simulink model "model_compatible"  (Simulink 7.5)
(part 8 of 10)

      | %<Name>
  bus795 : powerlib/Measurements/Load Flow Bus  LConnTagsString=a  Phases=single  Connectors=on one side  ID=bus795  Vbase=380000  Vref=1  Vangle=0  VLF=1  VLFb=1  VLFc=1  angleLF=0  angleLFb=0  angleLFc=0
      settings: AttributesFormatString=|
      | %<ID>
      | %<Vbase>V
      | %<VLF>pu
      | %<angleLF>deg.
      | %<Name>
  bus796 : powerlib/Measurements/Load Flow Bus  LConnTagsString=a  Phases=single  Connectors=on one side  ID=bus796  Vbase=380000  Vref=1  Vangle=0  VLF=1  VLFb=1  VLFc=1  angleLF=0  angleLFb=0  angleLFc=0
      settings: AttributesFormatString=|
      | %<ID>
      | %<Vbase>V
      | %<VLF>pu
      | %<angleLF>deg.
      | %<Name>
  bus797 : powerlib/Measurements/Load Flow Bus  LConnTagsString=a  Phases=single  Connectors=on one side  ID=bus797  Vbase=380000  Vref=1  Vangle=0  VLF=1  VLFb=1  VLFc=1  angleLF=0  angleLFb=0  angleLFc=0
      settings: AttributesFormatString=|
      | %<ID>
      | %<Vbase>V
      | %<VLF>pu
      | %<angleLF>deg.
      | %<Name>
  bus798 : powerlib/Measurements/Load Flow Bus  LConnTagsString=a  Phases=single  Connectors=on one side  ID=bus798  Vbase=380000  Vref=1  Vangle=0  VLF=1  VLFb=1  VLFc=1  angleLF=0  angleLFb=0  angleLFc=0
      settings: AttributesFormatString=|
      | %<ID>
      | %<Vbase>V
      | %<VLF>pu
      | %<angleLF>deg.
      | %<Name>
  bus799 : powerlib/Measurements/Load Flow Bus  LConnTagsString=a  Phases=single  Connectors=on one side  ID=bus799  Vbase=380000  Vref=1  Vangle=0  VLF=1  VLFb=1  VLFc=1  angleLF=0  angleLFb=0  angleLFc=0
      settings: AttributesFormatString=|
      | %<ID>
      | %<Vbase>V
      | %<VLF>pu
      | %<angleLF>deg.
      | %<Name>
  bus8 : powerlib/Measurements/Load Flow Bus  LConnTagsString=a  Phases=single  Connectors=on one side  ID=bus8  Vbase=220000  Vref=1  Vangle=0  VLF=1  VLFb=1  VLFc=1  angleLF=0  angleLFb=0  angleLFc=0
      settings: AttributesFormatString=|
      | %<ID>
      | %<Vbase>V
      | %<VLF>pu
      | %<angleLF>deg.
      | %<Name>
  bus80 : powerlib/Measurements/Load Flow Bus  LConnTagsString=a  Phases=single  Connectors=on one side  ID=bus80  Vbase=220000  Vref=1  Vangle=0  VLF=1  VLFb=1  VLFc=1  angleLF=0  angleLFb=0  angleLFc=0
      settings: AttributesFormatString=|
      | %<ID>
      | %<Vbase>V
      | %<VLF>pu
      | %<angleLF>deg.
      | %<Name>
  bus800 : powerlib/Measurements/Load Flow Bus  LConnTagsString=a  Phases=single  Connectors=on one side  ID=bus800  Vbase=380000  Vref=1  Vangle=0  VLF=1  VLFb=1  VLFc=1  angleLF=0  angleLFb=0  angleLFc=0
      settings: AttributesFormatString=|
      | %<ID>
      | %<Vbase>V
      | %<VLF>pu
      | %<angleLF>deg.
      | %<Name>
  bus801 : powerlib/Measurements/Load Flow Bus  LConnTagsString=a  Phases=single  Connectors=on one side  ID=bus801  Vbase=380000  Vref=1  Vangle=0  VLF=1  VLFb=1  VLFc=1  angleLF=0  angleLFb=0  angleLFc=0
      settings: AttributesFormatString=|
      | %<ID>
      | %<Vbase>V
      | %<VLF>pu
      | %<angleLF>deg.
      | %<Name>
  bus802 : powerlib/Measurements/Load Flow Bus  LConnTagsString=a  Phases=single  Connectors=on one side  ID=bus802  Vbase=380000  Vref=1  Vangle=0  VLF=1  VLFb=1  VLFc=1  angleLF=0  angleLFb=0  angleLFc=0
      settings: AttributesFormatString=|
      | %<ID>
      | %<Vbase>V
      | %<VLF>pu
      | %<angleLF>deg.
      | %<Name>
  bus803 : powerlib/Measurements/Load Flow Bus  LConnTagsString=a  Phases=single  Connectors=on one side  ID=bus803  Vbase=380000  Vref=1  Vangle=0  VLF=1  VLFb=1  VLFc=1  angleLF=0  angleLFb=0  angleLFc=0
      settings: AttributesFormatString=|
      | %<ID>
      | %<Vbase>V
      | %<VLF>pu
      | %<angleLF>deg.
      | %<Name>
  bus804 : powerlib/Measurements/Load Flow Bus  LConnTagsString=a  Phases=single  Connectors=on one side  ID=bus804  Vbase=380000  Vref=1  Vangle=0  VLF=1  VLFb=1  VLFc=1  angleLF=0  angleLFb=0  angleLFc=0
      settings: AttributesFormatString=|
      | %<ID>
      | %<Vbase>V
      | %<VLF>pu
      | %<angleLF>deg.
      | %<Name>
  bus805 : powerlib/Measurements/Load Flow Bus  LConnTagsString=a  Phases=single  Connectors=on one side  ID=bus805  Vbase=380000  Vref=1  Vangle=0  VLF=1  VLFb=1  VLFc=1  angleLF=0  angleLFb=0  angleLFc=0
      settings: AttributesFormatString=|
      | %<ID>
      | %<Vbase>V
      | %<VLF>pu
      | %<angleLF>deg.
      | %<Name>
  bus806 : powerlib/Measurements/Load Flow Bus  LConnTagsString=a  Phases=single  Connectors=on one side  ID=bus806  Vbase=380000  Vref=1  Vangle=0  VLF=1  VLFb=1  VLFc=1  angleLF=0  angleLFb=0  angleLFc=0
      settings: AttributesFormatString=|
      | %<ID>
      | %<Vbase>V
      | %<VLF>pu
      | %<angleLF>deg.
      | %<Name>
  bus807 : powerlib/Measurements/Load Flow Bus  LConnTagsString=a  Phases=single  Connectors=on one side  ID=bus807  Vbase=380000  Vref=1  Vangle=0  VLF=1  VLFb=1  VLFc=1  angleLF=0  angleLFb=0  angleLFc=0
      settings: AttributesFormatString=|
      | %<ID>
      | %<Vbase>V
      | %<VLF>pu
      | %<angleLF>deg.
      | %<Name>
  bus808 : powerlib/Measurements/Load Flow Bus  LConnTagsString=a  Phases=single  Connectors=on one side  ID=bus808  Vbase=380000  Vref=1  Vangle=0  VLF=1  VLFb=1  VLFc=1  angleLF=0  angleLFb=0  angleLFc=0
      settings: AttributesFormatString=|
      | %<ID>
      | %<Vbase>V
      | %<VLF>pu
      | %<angleLF>deg.
      | %<Name>
  bus809 : powerlib/Measurements/Load Flow Bus  LConnTagsString=a  Phases=single  Connectors=on one side  ID=bus809  Vbase=132000  Vref=1  Vangle=0  VLF=1  VLFb=1  VLFc=1  angleLF=0  angleLFb=0  angleLFc=0
      settings: AttributesFormatString=|
      | %<ID>
      | %<Vbase>V
      | %<VLF>pu
      | %<angleLF>deg.
      | %<Name>
  bus81 : powerlib/Measurements/Load Flow Bus  LConnTagsString=a  Phases=single  Connectors=on one side  ID=bus81  Vbase=220000  Vref=1  Vangle=0  VLF=1  VLFb=1  VLFc=1  angleLF=0  angleLFb=0  angleLFc=0
      settings: AttributesFormatString=|
      | %<ID>
      | %<Vbase>V
      | %<VLF>pu
      | %<angleLF>deg.
      | %<Name>
  bus810 : powerlib/Measurements/Load Flow Bus  LConnTagsString=a  Phases=single  Connectors=on one side  ID=bus810  Vbase=380000  Vref=1  Vangle=0  VLF=1  VLFb=1  VLFc=1  angleLF=0  angleLFb=0  angleLFc=0
      settings: AttributesFormatString=|
      | %<ID>
      | %<Vbase>V
      | %<VLF>pu
      | %<angleLF>deg.
      | %<Name>
  bus811 : powerlib/Measurements/Load Flow Bus  LConnTagsString=a  Phases=single  Connectors=on one side  ID=bus811  Vbase=380000  Vref=1  Vangle=0  VLF=1  VLFb=1  VLFc=1  angleLF=0  angleLFb=0  angleLFc=0
      settings: AttributesFormatString=|
      | %<ID>
      | %<Vbase>V
      | %<VLF>pu
      | %<angleLF>deg.
      | %<Name>
  bus812 : powerlib/Measurements/Load Flow Bus  LConnTagsString=a  Phases=single  Connectors=on one side  ID=bus812  Vbase=380000  Vref=1  Vangle=0  VLF=1  VLFb=1  VLFc=1  angleLF=0  angleLFb=0  angleLFc=0
      settings: AttributesFormatString=|
      | %<ID>
      | %<Vbase>V
      | %<VLF>pu
      | %<angleLF>deg.
      | %<Name>
  bus813 : powerlib/Measurements/Load Flow Bus  LConnTagsString=a  Phases=single  Connectors=on one side  ID=bus813  Vbase=380000  Vref=1  Vangle=0  VLF=1  VLFb=1  VLFc=1  angleLF=0  angleLFb=0  angleLFc=0
      settings: AttributesFormatString=|
      | %<ID>
      | %<Vbase>V
      | %<VLF>pu
      | %<angleLF>deg.
      | %<Name>
  bus814 : powerlib/Measurements/Load Flow Bus  LConnTagsString=a  Phases=single  Connectors=on one side  ID=bus814  Vbase=380000  Vref=1  Vangle=0  VLF=1  VLFb=1  VLFc=1  angleLF=0  angleLFb=0  angleLFc=0
      settings: AttributesFormatString=|
      | %<ID>
      | %<Vbase>V
      | %<VLF>pu
      | %<angleLF>deg.
      | %<Name>
  bus815 : powerlib/Measurements/Load Flow Bus  LConnTagsString=a  Phases=single  Connectors=on one side  ID=bus815  Vbase=380000  Vref=1  Vangle=0  VLF=1  VLFb=1  VLFc=1  angleLF=0  angleLFb=0  angleLFc=0
      settings: AttributesFormatString=|
      | %<ID>
      | %<Vbase>V
      | %<VLF>pu
      | %<angleLF>deg.
      | %<Name>
  bus816 : powerlib/Measurements/Load Flow Bus  LConnTagsString=a  Phases=single  Connectors=on one side  ID=bus816  Vbase=380000  Vref=1  Vangle=0  VLF=1  VLFb=1  VLFc=1  angleLF=0  angleLFb=0  angleLFc=0
      settings: AttributesFormatString=|
      | %<ID>
      | %<Vbase>V
      | %<VLF>pu
      | %<angleLF>deg.
      | %<Name>
  bus817 : powerlib/Measurements/Load Flow Bus  LConnTagsString=a  Phases=single  Connectors=on one side  ID=bus817  Vbase=380000  Vref=1  Vangle=0  VLF=1  VLFb=1  VLFc=1  angleLF=0  angleLFb=0  angleLFc=0
      settings: AttributesFormatString=|
      | %<ID>
      | %<Vbase>V
      | %<VLF>pu
      | %<angleLF>deg.
      | %<Name>
  bus818 : powerlib/Measurements/Load Flow Bus  LConnTagsString=a  Phases=single  Connectors=on one side  ID=bus818  Vbase=380000  Vref=1  Vangle=0  VLF=1  VLFb=1  VLFc=1  angleLF=0  angleLFb=0  angleLFc=0
      settings: AttributesFormatString=|
      | %<ID>
      | %<Vbase>V
      | %<VLF>pu
      | %<angleLF>deg.
      | %<Name>
  bus819 : powerlib/Measurements/Load Flow Bus  LConnTagsString=a  Phases=single  Connectors=on one side  ID=bus819  Vbase=380000  Vref=1  Vangle=0  VLF=1  VLFb=1  VLFc=1  angleLF=0  angleLFb=0  angleLFc=0
      settings: AttributesFormatString=|
      | %<ID>
      | %<Vbase>V
      | %<VLF>pu
      | %<angleLF>deg.
      | %<Name>
  bus82 : powerlib/Measurements/Load Flow Bus  LConnTagsString=a  Phases=single  Connectors=on one side  ID=bus82  Vbase=220000  Vref=1  Vangle=0  VLF=1  VLFb=1  VLFc=1  angleLF=0  angleLFb=0  angleLFc=0
      settings: AttributesFormatString=|
      | %<ID>
      | %<Vbase>V
      | %<VLF>pu
      | %<angleLF>deg.
      | %<Name>
  bus820 : powerlib/Measurements/Load Flow Bus  LConnTagsString=a  Phases=single  Connectors=on one side  ID=bus820  Vbase=380000  Vref=1  Vangle=0  VLF=1  VLFb=1  VLFc=1  angleLF=0  angleLFb=0  angleLFc=0
      settings: AttributesFormatString=|
      | %<ID>
      | %<Vbase>V
      | %<VLF>pu
      | %<angleLF>deg.
      | %<Name>
  bus821 : powerlib/Measurements/Load Flow Bus  LConnTagsString=a  Phases=single  Connectors=on one side  ID=bus821  Vbase=380000  Vref=1  Vangle=0  VLF=1  VLFb=1  VLFc=1  angleLF=0  angleLFb=0  angleLFc=0
      settings: AttributesFormatString=|
      | %<ID>
      | %<Vbase>V
      | %<VLF>pu
      | %<angleLF>deg.
      | %<Name>
  bus822 : powerlib/Measurements/Load Flow Bus  LConnTagsString=a  Phases=single  Connectors=on one side  ID=bus822  Vbase=380000  Vref=1  Vangle=0  VLF=1  VLFb=1  VLFc=1  angleLF=0  angleLFb=0  angleLFc=0
      settings: AttributesFormatString=|
      | %<ID>
      | %<Vbase>V
      | %<VLF>pu
      | %<angleLF>deg.
      | %<Name>
  bus823 : powerlib/Measurements/Load Flow Bus  LConnTagsString=a  Phases=single  Connectors=on one side  ID=bus823  Vbase=380000  Vref=1  Vangle=0  VLF=1  VLFb=1  VLFc=1  angleLF=0  angleLFb=0  angleLFc=0
      settings: AttributesFormatString=|
      | %<ID>
      | %<Vbase>V
      | %<VLF>pu
      | %<angleLF>deg.
      | %<Name>
  bus824 : powerlib/Measurements/Load Flow Bus  LConnTagsString=a  Phases=single  Connectors=on one side  ID=bus824  Vbase=380000  Vref=1  Vangle=0  VLF=1  VLFb=1  VLFc=1  angleLF=0  angleLFb=0  angleLFc=0
      settings: AttributesFormatString=|
      | %<ID>
      | %<Vbase>V
      | %<VLF>pu
      | %<angleLF>deg.
      | %<Name>
  bus825 : powerlib/Measurements/Load Flow Bus  LConnTagsString=a  Phases=single  Connectors=on one side  ID=bus825  Vbase=380000  Vref=1  Vangle=0  VLF=1  VLFb=1  VLFc=1  angleLF=0  angleLFb=0  angleLFc=0
      settings: AttributesFormatString=|
      | %<ID>
      | %<Vbase>V
      | %<VLF>pu
      | %<angleLF>deg.
      | %<Name>
  bus826 : powerlib/Measurements/Load Flow Bus  LConnTagsString=a  Phases=single  Connectors=on one side  ID=bus826  Vbase=380000  Vref=1  Vangle=0  VLF=1  VLFb=1  VLFc=1  angleLF=0  angleLFb=0  angleLFc=0
      settings: AttributesFormatString=|
      | %<ID>
      | %<Vbase>V
      | %<VLF>pu
      | %<angleLF>deg.
      | %<Name>
  bus827 : powerlib/Measurements/Load Flow Bus  LConnTagsString=a  Phases=single  Connectors=on one side  ID=bus827  Vbase=380000  Vref=1  Vangle=0  VLF=1  VLFb=1  VLFc=1  angleLF=0  angleLFb=0  angleLFc=0
      settings: AttributesFormatString=|
      | %<ID>
      | %<Vbase>V
      | %<VLF>pu
      | %<angleLF>deg.
      | %<Name>
  bus828 : powerlib/Measurements/Load Flow Bus  LConnTagsString=a  Phases=single  Connectors=on one side  ID=bus828  Vbase=380000  Vref=1  Vangle=0  VLF=1  VLFb=1  VLFc=1  angleLF=0  angleLFb=0  angleLFc=0
      settings: AttributesFormatString=|
      | %<ID>
      | %<Vbase>V
      | %<VLF>pu
      | %<angleLF>deg.
      | %<Name>
  bus829 : powerlib/Measurements/Load Flow Bus  LConnTagsString=a  Phases=single  Connectors=on one side  ID=bus829  Vbase=380000  Vref=1  Vangle=0  VLF=1  VLFb=1  VLFc=1  angleLF=0  angleLFb=0  angleLFc=0
      settings: AttributesFormatString=|
      | %<ID>
      | %<Vbase>V
      | %<VLF>pu
      | %<angleLF>deg.
      | %<Name>
  bus83 : powerlib/Measurements/Load Flow Bus  LConnTagsString=a  Phases=single  Connectors=on one side  ID=bus83  Vbase=220000  Vref=1  Vangle=0  VLF=1  VLFb=1  VLFc=1  angleLF=0  angleLFb=0  angleLFc=0
      settings: AttributesFormatString=|
      | %<ID>
      | %<Vbase>V
      | %<VLF>pu
      | %<angleLF>deg.
      | %<Name>
  bus830 : powerlib/Measurements/Load Flow Bus  LConnTagsString=a  Phases=single  Connectors=on one side  ID=bus830  Vbase=380000  Vref=1  Vangle=0  VLF=1  VLFb=1  VLFc=1  angleLF=0  angleLFb=0  angleLFc=0
      settings: AttributesFormatString=|
      | %<ID>
      | %<Vbase>V
      | %<VLF>pu
      | %<angleLF>deg.
      | %<Name>
  bus831 : powerlib/Measurements/Load Flow Bus  LConnTagsString=a  Phases=single  Connectors=on one side  ID=bus831  Vbase=380000  Vref=1  Vangle=0  VLF=1  VLFb=1  VLFc=1  angleLF=0  angleLFb=0  angleLFc=0
      settings: AttributesFormatString=|
      | %<ID>
      | %<Vbase>V
      | %<VLF>pu
      | %<angleLF>deg.
      | %<Name>
  bus832 : powerlib/Measurements/Load Flow Bus  LConnTagsString=a  Phases=single  Connectors=on one side  ID=bus832  Vbase=380000  Vref=1  Vangle=0  VLF=1  VLFb=1  VLFc=1  angleLF=0  angleLFb=0  angleLFc=0
      settings: AttributesFormatString=|
      | %<ID>
      | %<Vbase>V
      | %<VLF>pu
      | %<angleLF>deg.
      | %<Name>
  bus833 : powerlib/Measurements/Load Flow Bus  LConnTagsString=a  Phases=single  Connectors=on one side  ID=bus833  Vbase=380000  Vref=1  Vangle=0  VLF=1  VLFb=1  VLFc=1  angleLF=0  angleLFb=0  angleLFc=0
      settings: AttributesFormatString=|
      | %<ID>
      | %<Vbase>V
      | %<VLF>pu
      | %<angleLF>deg.
      | %<Name>
  bus834 : powerlib/Measurements/Load Flow Bus  LConnTagsString=a  Phases=single  Connectors=on one side  ID=bus834  Vbase=380000  Vref=1  Vangle=0  VLF=1  VLFb=1  VLFc=1  angleLF=0  angleLFb=0  angleLFc=0
      settings: AttributesFormatString=|
      | %<ID>
      | %<Vbase>V
      | %<VLF>pu
      | %<angleLF>deg.
      | %<Name>
  bus835 : powerlib/Measurements/Load Flow Bus  LConnTagsString=a  Phases=single  Connectors=on one side  ID=bus835  Vbase=380000  Vref=1  Vangle=0  VLF=1  VLFb=1  VLFc=1  angleLF=0  angleLFb=0  angleLFc=0
      settings: AttributesFormatString=|
      | %<ID>
      | %<Vbase>V
      | %<VLF>pu
      | %<angleLF>deg.
      | %<Name>
  bus836 : powerlib/Measurements/Load Flow Bus  LConnTagsString=a  Phases=single  Connectors=on one side  ID=bus836  Vbase=380000  Vref=1  Vangle=0  VLF=1  VLFb=1  VLFc=1  angleLF=0  angleLFb=0  angleLFc=0
      settings: AttributesFormatString=|
      | %<ID>
      | %<Vbase>V
      | %<VLF>pu
      | %<angleLF>deg.
      | %<Name>
  bus837 : powerlib/Measurements/Load Flow Bus  LConnTagsString=a  Phases=single  Connectors=on one side  ID=bus837  Vbase=380000  Vref=1  Vangle=0  VLF=1  VLFb=1  VLFc=1  angleLF=0  angleLFb=0  angleLFc=0
      settings: AttributesFormatString=|
      | %<ID>
      | %<Vbase>V
      | %<VLF>pu
      | %<angleLF>deg.
      | %<Name>
  bus838 : powerlib/Measurements/Load Flow Bus  LConnTagsString=a  Phases=single  Connectors=on one side  ID=bus838  Vbase=380000  Vref=1  Vangle=0  VLF=1  VLFb=1  VLFc=1  angleLF=0  angleLFb=0  angleLFc=0
      settings: AttributesFormatString=|
      | %<ID>
      | %<Vbase>V
      | %<VLF>pu
      | %<angleLF>deg.
      | %<Name>
  bus839 : powerlib/Measurements/Load Flow Bus  LConnTagsString=a  Phases=single  Connectors=on one side  ID=bus839  Vbase=380000  Vref=1  Vangle=0  VLF=1  VLFb=1  VLFc=1  angleLF=0  angleLFb=0  angleLFc=0
      settings: AttributesFormatString=|
      | %<ID>
      | %<Vbase>V
      | %<VLF>pu
      | %<angleLF>deg.
      | %<Name>
  bus84 : powerlib/Measurements/Load Flow Bus  LConnTagsString=a  Phases=single  Connectors=on one side  ID=bus84  Vbase=220000  Vref=1  Vangle=0  VLF=1  VLFb=1  VLFc=1  angleLF=0  angleLFb=0  angleLFc=0
      settings: AttributesFormatString=|
      | %<ID>
      | %<Vbase>V
      | %<VLF>pu
      | %<angleLF>deg.
      | %<Name>
  bus840 : powerlib/Measurements/Load Flow Bus  LConnTagsString=a  Phases=single  Connectors=on one side  ID=bus840  Vbase=380000  Vref=1  Vangle=0  VLF=1  VLFb=1  VLFc=1  angleLF=0  angleLFb=0  angleLFc=0
      settings: AttributesFormatString=|
      | %<ID>
      | %<Vbase>V
      | %<VLF>pu
      | %<angleLF>deg.
      | %<Name>
  bus841 : powerlib/Measurements/Load Flow Bus  LConnTagsString=a  Phases=single  Connectors=on one side  ID=bus841  Vbase=380000  Vref=1  Vangle=0  VLF=1  VLFb=1  VLFc=1  angleLF=0  angleLFb=0  angleLFc=0
      settings: AttributesFormatString=|
      | %<ID>
      | %<Vbase>V
      | %<VLF>pu
      | %<angleLF>deg.
      | %<Name>
  bus842 : powerlib/Measurements/Load Flow Bus  LConnTagsString=a  Phases=single  Connectors=on one side  ID=bus842  Vbase=380000  Vref=1  Vangle=0  VLF=1  VLFb=1  VLFc=1  angleLF=0  angleLFb=0  angleLFc=0
      settings: AttributesFormatString=|
      | %<ID>
      | %<Vbase>V
      | %<VLF>pu
      | %<angleLF>deg.
      | %<Name>
  bus843 : powerlib/Measurements/Load Flow Bus  LConnTagsString=a  Phases=single  Connectors=on one side  ID=bus843  Vbase=380000  Vref=1  Vangle=0  VLF=1  VLFb=1  VLFc=1  angleLF=0  angleLFb=0  angleLFc=0
      settings: AttributesFormatString=|
      | %<ID>
      | %<Vbase>V
      | %<VLF>pu
      | %<angleLF>deg.
      | %<Name>
  bus844 : powerlib/Measurements/Load Flow Bus  LConnTagsString=a  Phases=single  Connectors=on one side  ID=bus844  Vbase=380000  Vref=1  Vangle=0  VLF=1  VLFb=1  VLFc=1  angleLF=0  angleLFb=0  angleLFc=0
      settings: AttributesFormatString=|
      | %<ID>
      | %<Vbase>V
      | %<VLF>pu
      | %<angleLF>deg.
      | %<Name>
  bus845 : powerlib/Measurements/Load Flow Bus  LConnTagsString=a  Phases=single  Connectors=on one side  ID=bus845  Vbase=380000  Vref=1  Vangle=0  VLF=1  VLFb=1  VLFc=1  angleLF=0  angleLFb=0  angleLFc=0
      settings: AttributesFormatString=|
      | %<ID>
      | %<Vbase>V
      | %<VLF>pu
      | %<angleLF>deg.
      | %<Name>
  bus846 : powerlib/Measurements/Load Flow Bus  LConnTagsString=a  Phases=single  Connectors=on one side  ID=bus846  Vbase=380000  Vref=1  Vangle=0  VLF=1  VLFb=1  VLFc=1  angleLF=0  angleLFb=0  angleLFc=0
      settings: AttributesFormatString=|
      | %<ID>
      | %<Vbase>V
      | %<VLF>pu
      | %<angleLF>deg.
      | %<Name>
  bus85 : powerlib/Measurements/Load Flow Bus  LConnTagsString=a  Phases=single  Connectors=on one side  ID=bus85  Vbase=220000  Vref=1  Vangle=0  VLF=1  VLFb=1  VLFc=1  angleLF=0  angleLFb=0  angleLFc=0
      settings: AttributesFormatString=|
      | %<ID>
      | %<Vbase>V
      | %<VLF>pu
      | %<angleLF>deg.
      | %<Name>
  bus86 : powerlib/Measurements/Load Flow Bus  LConnTagsString=a  Phases=single  Connectors=on one side  ID=bus86  Vbase=220000  Vref=1  Vangle=0  VLF=1  VLFb=1  VLFc=1  angleLF=0  angleLFb=0  angleLFc=0
      settings: AttributesFormatString=|
      | %<ID>
      | %<Vbase>V
      | %<VLF>pu
      | %<angleLF>deg.
      | %<Name>
  bus87 : powerlib/Measurements/Load Flow Bus  LConnTagsString=a  Phases=single  Connectors=on one side  ID=bus87  Vbase=220000  Vref=1  Vangle=0  VLF=1  VLFb=1  VLFc=1  angleLF=0  angleLFb=0  angleLFc=0
      settings: AttributesFormatString=|
      | %<ID>
      | %<Vbase>V
      | %<VLF>pu
      | %<angleLF>deg.
      | %<Name>
  bus88 : powerlib/Measurements/Load Flow Bus  LConnTagsString=a  Phases=single  Connectors=on one side  ID=bus88  Vbase=220000  Vref=1  Vangle=0  VLF=1  VLFb=1  VLFc=1  angleLF=0  angleLFb=0  angleLFc=0
      settings: AttributesFormatString=|
      | %<ID>
      | %<Vbase>V
      | %<VLF>pu
      | %<angleLF>deg.
      | %<Name>
  bus89 : powerlib/Measurements/Load Flow Bus  LConnTagsString=a  Phases=single  Connectors=on one side  ID=bus89  Vbase=220000  Vref=1  Vangle=0  VLF=1  VLFb=1  VLFc=1  angleLF=0  angleLFb=0  angleLFc=0
      settings: AttributesFormatString=|
      | %<ID>
      | %<Vbase>V
      | %<VLF>pu
      | %<angleLF>deg.
      | %<Name>
  bus9 : powerlib/Measurements/Load Flow Bus  LConnTagsString=a  Phases=single  Connectors=on one side  ID=bus9  Vbase=220000  Vref=1  Vangle=0  VLF=1  VLFb=1  VLFc=1  angleLF=0  angleLFb=0  angleLFc=0
      settings: AttributesFormatString=|
      | %<ID>
      | %<Vbase>V
      | %<VLF>pu
      | %<angleLF>deg.
      | %<Name>
  bus90 : powerlib/Measurements/Load Flow Bus  LConnTagsString=a  Phases=single  Connectors=on one side  ID=bus90  Vbase=220000  Vref=1  Vangle=0  VLF=1  VLFb=1  VLFc=1  angleLF=0  angleLFb=0  angleLFc=0
      settings: AttributesFormatString=|
      | %<ID>
      | %<Vbase>V
      | %<VLF>pu
      | %<angleLF>deg.
      | %<Name>
  bus91 : powerlib/Measurements/Load Flow Bus  LConnTagsString=a  Phases=single  Connectors=on one side  ID=bus91  Vbase=220000  Vref=1  Vangle=0  VLF=1  VLFb=1  VLFc=1  angleLF=0  angleLFb=0  angleLFc=0
      settings: AttributesFormatString=|
      | %<ID>
      | %<Vbase>V
      | %<VLF>pu
      | %<angleLF>deg.
      | %<Name>
  bus92 : powerlib/Measurements/Load Flow Bus  LConnTagsString=a  Phases=single  Connectors=on one side  ID=bus92  Vbase=220000  Vref=1  Vangle=0  VLF=1  VLFb=1  VLFc=1  angleLF=0  angleLFb=0  angleLFc=0
      settings: AttributesFormatString=|
      | %<ID>
      | %<Vbase>V
      | %<VLF>pu
      | %<angleLF>deg.
      | %<Name>
  bus93 : powerlib/Measurements/Load Flow Bus  LConnTagsString=a  Phases=single  Connectors=on one side  ID=bus93  Vbase=220000  Vref=1  Vangle=0  VLF=1  VLFb=1  VLFc=1  angleLF=0  angleLFb=0  angleLFc=0
      settings: AttributesFormatString=|
      | %<ID>
      | %<Vbase>V
      | %<VLF>pu
      | %<angleLF>deg.
      | %<Name>
  bus94 : powerlib/Measurements/Load Flow Bus  LConnTagsString=a  Phases=single  Connectors=on one side  ID=bus94  Vbase=220000  Vref=1  Vangle=0  VLF=1  VLFb=1  VLFc=1  angleLF=0  angleLFb=0  angleLFc=0
      settings: AttributesFormatString=|
      | %<ID>
      | %<Vbase>V
      | %<VLF>pu
      | %<angleLF>deg.
      | %<Name>
  bus95 : powerlib/Measurements/Load Flow Bus  LConnTagsString=a  Phases=single  Connectors=on one side  ID=bus95  Vbase=220000  Vref=1  Vangle=0  VLF=1  VLFb=1  VLFc=1  angleLF=0  angleLFb=0  angleLFc=0
      settings: AttributesFormatString=|
      | %<ID>
      | %<Vbase>V
      | %<VLF>pu
      | %<angleLF>deg.
      | %<Name>
  bus96 : powerlib/Measurements/Load Flow Bus  LConnTagsString=a  Phases=single  Connectors=on one side  ID=bus96  Vbase=220000  Vref=1  Vangle=0  VLF=1  VLFb=1  VLFc=1  angleLF=0  angleLFb=0  angleLFc=0
      settings: AttributesFormatString=|
      | %<ID>
      | %<Vbase>V
      | %<VLF>pu
      | %<angleLF>deg.
      | %<Name>
  bus97 : powerlib/Measurements/Load Flow Bus  LConnTagsString=a  Phases=single  Connectors=on one side  ID=bus97  Vbase=220000  Vref=1  Vangle=0  VLF=1  VLFb=1  VLFc=1  angleLF=0  angleLFb=0  angleLFc=0
      settings: AttributesFormatString=|
      | %<ID>
      | %<Vbase>V
      | %<VLF>pu
      | %<angleLF>deg.
      | %<Name>
  bus98 : powerlib/Measurements/Load Flow Bus  LConnTagsString=a  Phases=single  Connectors=on one side  ID=bus98  Vbase=220000  Vref=1  Vangle=0  VLF=1  VLFb=1  VLFc=1  angleLF=0  angleLFb=0  angleLFc=0
      settings: AttributesFormatString=|
      | %<ID>
      | %<Vbase>V
      | %<VLF>pu
      | %<angleLF>deg.
      | %<Name>
  bus99 : powerlib/Measurements/Load Flow Bus  LConnTagsString=a  Phases=single  Connectors=on one side  ID=bus99  Vbase=220000  Vref=1  Vangle=0  VLF=1  VLFb=1  VLFc=1  angleLF=0  angleLFb=0  angleLFc=0
      settings: AttributesFormatString=|
      | %<ID>
      | %<Vbase>V
      | %<VLF>pu
      | %<angleLF>deg.
      | %<Name>
  derivazione_Dalmine_CN_166196787_220000_CN_68299044_220000 : powerlib/Elements/Distributed Parameters Line  Phases=3  Frequency=50  Resistance=[0.01273 0.3864]  Inductance="[0.9337e-3  4.1264e-3]"  Capacitance=[12.74e-9 7.751e-9]  Length=30.2075  x1=[8.73114913702011e-11 380000 380000;314.159265358979 314.159265358979 314.159265358979;-0.177670123217348 0.415246442777429 -1.15554988401747]  x2=[1.26090477118469e-09 381852.398472139 381852.398472139;314.159265358979 314.159265358979 314.159265358979;-1.41941675517191 0.415007521738739 -1.15578880505616]  x3=[1.07663708898761e-11 1405.24743813465 1405.24743813466;314.159265358979 314.159265358979 314.159265358979;-2.70558821102223 0.316110507002444 -1.25468581979246]  x4=[8.62234243168895e-12 1405.96374414071 1405.9637441407;314.159265358979 314.159265358979 314.159265358979;0.245769282942371 0.405640215255436 -1.16515611153945]  x5=0.000565541566995742  V1=ones(3,3)  V2=ones(3,3)  I1=ones(3,3)  I2=ones(3,3)  nHarmo=1  Measurements=None
  powergui : powerlib/powergui  Priority=1  SimulationMode=Phasor  SolverType=Tustin/Backward Euler (TBE)  SampleTime=50e-6  frequency=50  SPID=off  DisableSnubberDevices=off  DisableRonSwitches=off  DisableVfSwitches=off  SwTol=0  DisplayEquations=off  Interpol=off  ExternalGateDelay=off  methode=off  Ts=10  FunctionMessages=off  echomessages=off  HookPort=off  EnableUseOfTLC=off  x0status=blocks  frequencyindice=50  Pbase=3000e6  ErrMax=0.0001  Iterations=50  UnitsV=V  UnitsW=W  buscounter=0  RestoreLinks=warning  ResistiveCurrentMeasurement=off  Frange=[0:2:500]  Ylog=off  Xlog=on  ShowGrid=off  save=off  variable=ZData  structure=0  ZoomFFT=off  StartTime=0.0  cycles=1  DisplayStyle=1  fundamental=60  FreqAxis=off  MaxFrequency=1000  frequencyindicesteady=1  RmsSteady=1  display=off
  connections:
  San_Pancrazio_Lana_CN_152457216_220000_CN_42862642_220000/LConn1 -- T_152457216_220000_San_Pancrazio/LConn1 -- San_Pancrazio_Lana_CN_152457216_220000_CN_96727258_220000/LConn1 -- San_Pancrazio_Lana_CN_152457216_220000_CN_153548074_220000/LConn1
  San_Pancrazio_Lana_CN_152457216_220000_CN_42862642_220000/LConn2 -- T_152457216_220000_San_Pancrazio/LConn2 -- San_Pancrazio_Lana_CN_152457216_220000_CN_96727258_220000/LConn2 -- San_Pancrazio_Lana_CN_152457216_220000_CN_153548074_220000/LConn2
  San_Pancrazio_Lana_CN_152457216_220000_CN_42862642_220000/LConn3 -- T_152457216_220000_San_Pancrazio/LConn3 -- San_Pancrazio_Lana_CN_152457216_220000_CN_96727258_220000/LConn3 -- bus1/LConn1 -- San_Pancrazio_Lana_CN_152457216_220000_CN_153548074_220000/LConn3
  San_Pancrazio_Lana_CN_152457216_220000_CN_42862642_220000/RConn1 -- T_42862642_220000_Lana/LConn1 -- Lana_Sant'Antonio_CN_42862642_220000_CN_105827045_220000/LConn1 -- Lana_Sant'Antonio_CN_42862642_220000_CN_105801489_220000/LConn1 -- Lana_Sant'Antonio_CN_42862642_220000_CN_147466201_220000/LConn1
  San_Pancrazio_Lana_CN_152457216_220000_CN_42862642_220000/RConn2 -- T_42862642_220000_Lana/LConn2 -- Lana_Sant'Antonio_CN_42862642_220000_CN_105827045_220000/LConn2 -- Lana_Sant'Antonio_CN_42862642_220000_CN_105801489_220000/LConn2 -- Lana_Sant'Antonio_CN_42862642_220000_CN_147466201_220000/LConn2
  San_Pancrazio_Lana_CN_152457216_220000_CN_42862642_220000/RConn3 -- T_42862642_220000_Lana/LConn3 -- Lana_Sant'Antonio_CN_42862642_220000_CN_105827045_220000/LConn3 -- Lana_Sant'Antonio_CN_42862642_220000_CN_105801489_220000/LConn3 -- Lana_Sant'Antonio_CN_42862642_220000_CN_147466201_220000/LConn3 -- bus2/LConn1
  T_153548074_220000_Castelbello/LConn1 -- San_Pancrazio_Lana_CN_152457216_220000_CN_153548074_220000/RConn1
  T_153548074_220000_Castelbello/LConn2 -- San_Pancrazio_Lana_CN_152457216_220000_CN_153548074_220000/RConn2
  San_Pancrazio_Lana_CN_152457216_220000_CN_153548074_220000/RConn3 -- T_153548074_220000_Castelbello/LConn3 -- bus3/LConn1
  T_96727258_220000_Eppan___Appiano/LConn1 -- San_Pancrazio_Lana_CN_152457216_220000_CN_96727258_220000/RConn1
  T_96727258_220000_Eppan___Appiano/LConn2 -- San_Pancrazio_Lana_CN_152457216_220000_CN_96727258_220000/RConn2
  San_Pancrazio_Lana_CN_152457216_220000_CN_96727258_220000/RConn3 -- T_96727258_220000_Eppan___Appiano/LConn3 -- bus4/LConn1
  T_205597560_220000_/LConn1 -- Mincio_Marcaria_CN_205597560_220000_CN103562617/LConn1
  T_205597560_220000_/LConn2 -- Mincio_Marcaria_CN_205597560_220000_CN103562617/LConn2
  Mincio_Marcaria_CN_205597560_220000_CN103562617/LConn3 -- T_205597560_220000_/LConn3 -- bus5/LConn1
  Mincio_Marcaria_CN_205597560_220000_CN103562617/RConn1 -- G_103562617_Centrale_del_Mincio/RConn1 -- Mincio_Marcaria_CN_163058980_220000_CN103562617/LConn1
  Mincio_Marcaria_CN_205597560_220000_CN103562617/RConn2 -- G_103562617_Centrale_del_Mincio/RConn2 -- Mincio_Marcaria_CN_163058980_220000_CN103562617/LConn2
  Mincio_Marcaria_CN_205597560_220000_CN103562617/RConn3 -- G_103562617_Centrale_del_Mincio/RConn3 -- Mincio_Marcaria_CN_163058980_220000_CN103562617/LConn3 -- bus6/LConn1
  Avise_Villeneuve_CN_102675884_220000_CN_102185362_220000/LConn1 -- T_102675884_220000_Avise/LConn1 -- _CN_102675884_220000_CN_103127416_220000/LConn1
  Avise_Villeneuve_CN_102675884_220000_CN_102185362_220000/LConn2 -- T_102675884_220000_Avise/LConn2 -- _CN_102675884_220000_CN_103127416_220000/LConn2
  Avise_Villeneuve_CN_102675884_220000_CN_102185362_220000/LConn3 -- T_102675884_220000_Avise/LConn3 -- _CN_102675884_220000_CN_103127416_220000/LConn3 -- bus7/LConn1
  Avise_Villeneuve_CN_102675884_220000_CN_102185362_220000/RConn1 -- T_102185362_220000_Villeneuve/LConn1 -- _CN_103007030_220000_CN_102185362_220000/LConn1 -- Villeneuve_Villa_CN_102185356_220000_CN_102185362_220000/LConn1
  Avise_Villeneuve_CN_102675884_220000_CN_102185362_220000/RConn2 -- T_102185362_220000_Villeneuve/LConn2 -- _CN_103007030_220000_CN_102185362_220000/LConn2 -- Villeneuve_Villa_CN_102185356_220000_CN_102185362_220000/LConn2
  Avise_Villeneuve_CN_102675884_220000_CN_102185362_220000/RConn3 -- T_102185362_220000_Villeneuve/LConn3 -- _CN_103007030_220000_CN_102185362_220000/LConn3 -- Villeneuve_Villa_CN_102185356_220000_CN_102185362_220000/LConn3 -- bus8/LConn1
  T_103127416_220000_Valpelline_G1/LConn1 -- _CN_102675884_220000_CN_103127416_220000/RConn1
  T_103127416_220000_Valpelline_G1/LConn2 -- _CN_102675884_220000_CN_103127416_220000/RConn2
  _CN_102675884_220000_CN_103127416_220000/RConn3 -- T_103127416_220000_Valpelline_G1/LConn3 -- bus9/LConn1
  _CN_132723724_220000_CN_376502663_220000/LConn1 -- T_132723724__/LConn1 -- Patria_Colli_Aminei_CN_132723724_220000_CN_114661587_220000/LConn1
  _CN_132723724_220000_CN_376502663_220000/LConn2 -- T_132723724__/LConn2 -- Patria_Colli_Aminei_CN_132723724_220000_CN_114661587_220000/LConn2
  _CN_132723724_220000_CN_376502663_220000/LConn3 -- T_132723724__/LConn3 -- Patria_Colli_Aminei_CN_132723724_220000_CN_114661587_220000/LConn3 -- bus10/LConn1
  _CN_132723724_220000_CN_376502663_220000/RConn1 -- T_376502663_220000_Colli_Aminei/LConn1 -- Colli_Aminei_Secondigliano_CN_377444657_220000_CN_376502663_220000/LConn1 -- Colli_Aminei_Arenella_CN_376502663_220000_CN_377588144_220000/LConn1
  _CN_132723724_220000_CN_376502663_220000/RConn2 -- T_376502663_220000_Colli_Aminei/LConn2 -- Colli_Aminei_Secondigliano_CN_377444657_220000_CN_376502663_220000/LConn2 -- Colli_Aminei_Arenella_CN_376502663_220000_CN_377588144_220000/LConn2
  _CN_132723724_220000_CN_376502663_220000/RConn3 -- T_376502663_220000_Colli_Aminei/LConn3 -- Colli_Aminei_Secondigliano_CN_377444657_220000_CN_376502663_220000/LConn3 -- Colli_Aminei_Arenella_CN_376502663_220000_CN_377588144_220000/LConn3 -- bus11/LConn1
  Patria_Colli_Aminei_CN_132723724_220000_CN_114661587_220000/RConn1 -- T_114661587_380000_Patria/RConn4 -- Patria_San_Antimo_CN_132455976_220000_CN_114661587_220000/LConn1 -- Astroni_Patria_CN_114661587_220000_CN_132725149_220000/LConn1 -- Patria_Pozzuoli_CN_114661587_220000_CN_132726160_220000/LConn1
  Patria_Colli_Aminei_CN_132723724_220000_CN_114661587_220000/RConn2 -- T_114661587_380000_Patria/RConn5 -- Patria_San_Antimo_CN_132455976_220000_CN_114661587_220000/LConn2 -- Astroni_Patria_CN_114661587_220000_CN_132725149_220000/LConn2 -- Patria_Pozzuoli_CN_114661587_220000_CN_132726160_220000/LConn2
  Patria_Colli_Aminei_CN_132723724_220000_CN_114661587_220000/RConn3 -- T_114661587_380000_Patria/RConn6 -- Patria_San_Antimo_CN_132455976_220000_CN_114661587_220000/LConn3 -- Astroni_Patria_CN_114661587_220000_CN_132725149_220000/LConn3 -- Patria_Pozzuoli_CN_114661587_220000_CN_132726160_220000/LConn3 -- bus12/LConn1
  Ercolano_San_Sebastiano_CN_202178573_220000_CN_132645607_220000/LConn1 -- T_202178573_220000_Ercolano/LConn1 -- Ercolano_San_Sebastiano_CN_202178573_220000_CN_132643428_220000/LConn1 -- Ercolano_San_Sebastiano_CN_202178573_220000_CN_202179060_220000/LConn1
  Ercolano_San_Sebastiano_CN_202178573_220000_CN_132645607_220000/LConn2 -- T_202178573_220000_Ercolano/LConn2 -- Ercolano_San_Sebastiano_CN_202178573_220000_CN_132643428_220000/LConn2 -- Ercolano_San_Sebastiano_CN_202178573_220000_CN_202179060_220000/LConn2
  Ercolano_San_Sebastiano_CN_202178573_220000_CN_132645607_220000/LConn3 -- T_202178573_220000_Ercolano/LConn3 -- Ercolano_San_Sebastiano_CN_202178573_220000_CN_132643428_220000/LConn3 -- Ercolano_San_Sebastiano_CN_202178573_220000_CN_202179060_220000/LConn3 -- bus13/LConn1
  T_132645607_220000_Torre_Nord/LConn1 -- Ercolano_San_Sebastiano_CN_202178573_220000_CN_132645607_220000/RConn1
  T_132645607_220000_Torre_Nord/LConn2 -- Ercolano_San_Sebastiano_CN_202178573_220000_CN_132645607_220000/RConn2
  Ercolano_San_Sebastiano_CN_202178573_220000_CN_132645607_220000/RConn3 -- T_132645607_220000_Torre_Nord/LConn3 -- bus14/LConn1
  T_132643428_220000_San_Valentino/LConn1 -- Ercolano_San_Sebastiano_CN_202178573_220000_CN_132643428_220000/RConn1
  T_132643428_220000_San_Valentino/LConn2 -- Ercolano_San_Sebastiano_CN_202178573_220000_CN_132643428_220000/RConn2
  Ercolano_San_Sebastiano_CN_202178573_220000_CN_132643428_220000/RConn3 -- T_132643428_220000_San_Valentino/LConn3 -- bus15/LConn1
  Ercolano_San_Sebastiano_CN_202178573_220000_CN_202179060_220000/RConn1 -- T_202179060_220000_San_Sebastiano/LConn1 -- San_Sebastiano_Castelluccia_CN_202179289_220000_CN_202179060_220000/LConn1
  Ercolano_San_Sebastiano_CN_202178573_220000_CN_202179060_220000/RConn2 -- T_202179060_220000_San_Sebastiano/LConn2 -- San_Sebastiano_Castelluccia_CN_202179289_220000_CN_202179060_220000/LConn2
  Ercolano_San_Sebastiano_CN_202178573_220000_CN_202179060_220000/RConn3 -- T_202179060_220000_San_Sebastiano/LConn3 -- San_Sebastiano_Castelluccia_CN_202179289_220000_CN_202179060_220000/LConn3 -- bus16/LConn1
  T_338969614_220000;150000_San_Filippo_del_Mela_gruppi_1,2,3,4/LConn1 -- _CN_338969614_220000_CN139107362/LConn1
  T_338969614_220000;150000_San_Filippo_del_Mela_gruppi_1,2,3,4/LConn2 -- _CN_338969614_220000_CN139107362/LConn2
  _CN_338969614_220000_CN139107362/LConn3 -- T_338969614_220000;150000_San_Filippo_del_Mela_gruppi_1,2,3,4/LConn3 -- bus17/LConn1
  _CN_338969614_220000_CN139107362/RConn1 -- G_139107362_Centrale_di_San_Filippo_del_Mela/RConn1 -- _CN_110140586_220000_CN139107362/LConn1 -- _CN_110138220_220000_CN139107362/LConn1
  _CN_338969614_220000_CN139107362/RConn2 -- G_139107362_Centrale_di_San_Filippo_del_Mela/RConn2 -- _CN_110140586_220000_CN139107362/LConn2 -- _CN_110138220_220000_CN139107362/LConn2
  _CN_338969614_220000_CN139107362/RConn3 -- G_139107362_Centrale_di_San_Filippo_del_Mela/RConn3 -- _CN_110140586_220000_CN139107362/LConn3 -- _CN_110138220_220000_CN139107362/LConn3 -- bus18/LConn1
  Trino_Nucleare_Balzola_CN_98427407_220000_CN_335012182_220000/LConn1 -- T_98427407_220000_Trino_220_kV/LConn1 -- Vercelli_Trino_CN_98427407_220000_CN_98638424_220000/LConn1 -- _CN_98427407_220000_CN95093082/LConn1
  Trino_Nucleare_Balzola_CN_98427407_220000_CN_335012182_220000/LConn2 -- T_98427407_220000_Trino_220_kV/LConn2 -- Vercelli_Trino_CN_98427407_220000_CN_98638424_220000/LConn2 -- _CN_98427407_220000_CN95093082/LConn2
  Trino_Nucleare_Balzola_CN_98427407_220000_CN_335012182_220000/LConn3 -- T_98427407_220000_Trino_220_kV/LConn3 -- Vercelli_Trino_CN_98427407_220000_CN_98638424_220000/LConn3 -- _CN_98427407_220000_CN95093082/LConn3 -- bus19/LConn1
  T_335012182_220000_Balzola_Stazione/LConn1 -- Trino_Nucleare_Balzola_CN_98427407_220000_CN_335012182_220000/RConn1
  T_335012182_220000_Balzola_Stazione/LConn2 -- Trino_Nucleare_Balzola_CN_98427407_220000_CN_335012182_220000/RConn2
  Trino_Nucleare_Balzola_CN_98427407_220000_CN_335012182_220000/RConn3 -- T_335012182_220000_Balzola_Stazione/LConn3 -- bus20/LConn1
  Vercelli_Trino_CN_98427407_220000_CN_98638424_220000/RConn1 -- T_98638424_220000_Vercelli_Nord/LConn1 -- Vercelli_Novara_Sud_CN_98638424_220000_CN_67461115_220000/LConn1
  Vercelli_Trino_CN_98427407_220000_CN_98638424_220000/RConn2 -- T_98638424_220000_Vercelli_Nord/LConn2 -- Vercelli_Novara_Sud_CN_98638424_220000_CN_67461115_220000/LConn2
  Vercelli_Trino_CN_98427407_220000_CN_98638424_220000/RConn3 -- T_98638424_220000_Vercelli_Nord/LConn3 -- Vercelli_Novara_Sud_CN_98638424_220000_CN_67461115_220000/LConn3 -- bus21/LConn1
  G_95093082_Ex_Centrale_Nucleare_di_Trino_Vercellese/RConn1 -- _CN_98427407_220000_CN95093082/RConn1
  G_95093082_Ex_Centrale_Nucleare_di_Trino_Vercellese/RConn2 -- _CN_98427407_220000_CN95093082/RConn2
  _CN_98427407_220000_CN95093082/RConn3 -- G_95093082_Ex_Centrale_Nucleare_di_Trino_Vercellese/RConn3 -- bus22/LConn1
  T_105462289_220000_Ponte/LConn1 -- Ponte_Verampio_CN_105462289_220000_CN_103418587_220000/LConn1
  T_105462289_220000_Ponte/LConn2 -- Ponte_Verampio_CN_105462289_220000_CN_103418587_220000/LConn2
  Ponte_Verampio_CN_105462289_220000_CN_103418587_220000/LConn3 -- T_105462289_220000_Ponte/LConn3 -- bus23/LConn1
  Ponte_Verampio_CN_105462289_220000_CN_103418587_220000/RConn1 -- T_103418587_220000_Verampio/LConn1 -- Pallanzeno_Verampio_CN_103418587_220000_CN_104114052_220000/LConn1
  Ponte_Verampio_CN_105462289_220000_CN_103418587_220000/RConn2 -- T_103418587_220000_Verampio/LConn2 -- Pallanzeno_Verampio_CN_103418587_220000_CN_104114052_220000/LConn2
  Ponte_Verampio_CN_105462289_220000_CN_103418587_220000/RConn3 -- T_103418587_220000_Verampio/LConn3 -- Pallanzeno_Verampio_CN_103418587_220000_CN_104114052_220000/LConn3 -- bus24/LConn1
  T_50589203_220000_Misterbianco/LConn1 -- Elettrodotto_Sorgente___Misterbianco_CN_50589203_220000_CN_110138220_220000/LConn1
  T_50589203_220000_Misterbianco/LConn2 -- Elettrodotto_Sorgente___Misterbianco_CN_50589203_220000_CN_110138220_220000/LConn2
  Elettrodotto_Sorgente___Misterbianco_CN_50589203_220000_CN_110138220_220000/LConn3 -- T_50589203_220000_Misterbianco/LConn3 -- bus25/LConn1
  Elettrodotto_Sorgente___Misterbianco_CN_50589203_220000_CN_110138220_220000/RConn1 -- T_110138220_380000_Sorgente/RConn4 -- Sorgente___Duferdofin_CN_194186027_220000_CN_110138220_220000/LConn1 -- _CN_110138220_220000_CN139107362/RConn1 -- Corriolo_Caracoli___Sorgente_CN_191960170_220000_CN_110138220_220000/LConn1
  Elettrodotto_Sorgente___Misterbianco_CN_50589203_220000_CN_110138220_220000/RConn2 -- T_110138220_380000_Sorgente/RConn5 -- Sorgente___Duferdofin_CN_194186027_220000_CN_110138220_220000/LConn2 -- _CN_110138220_220000_CN139107362/RConn2 -- Corriolo_Caracoli___Sorgente_CN_191960170_220000_CN_110138220_220000/LConn2
  Elettrodotto_Sorgente___Misterbianco_CN_50589203_220000_CN_110138220_220000/RConn3 -- T_110138220_380000_Sorgente/RConn6 -- Sorgente___Duferdofin_CN_194186027_220000_CN_110138220_220000/LConn3 -- _CN_110138220_220000_CN139107362/RConn3 -- bus26/LConn1 -- Corriolo_Caracoli___Sorgente_CN_191960170_220000_CN_110138220_220000/LConn3
  T_376642649_220000_Torretta/LConn1 -- _CN_376642649_220000_CN_79879307_220000/LConn1
  T_376642649_220000_Torretta/LConn2 -- _CN_376642649_220000_CN_79879307_220000/LConn2
  _CN_376642649_220000_CN_79879307_220000/LConn3 -- T_376642649_220000_Torretta/LConn3 -- bus27/LConn1
  _CN_376642649_220000_CN_79879307_220000/RConn1 -- T_79879307_220000_Sesto_San_Giovanni/LConn1 -- Brugherio_Sesto_CN_79879307_220000_CN_68299044_220000/LConn1 -- _CN_79879290_220000_CN_79879307_220000/LConn1
  _CN_376642649_220000_CN_79879307_220000/RConn2 -- T_79879307_220000_Sesto_San_Giovanni/LConn2 -- Brugherio_Sesto_CN_79879307_220000_CN_68299044_220000/LConn2 -- _CN_79879290_220000_CN_79879307_220000/LConn2
  _CN_376642649_220000_CN_79879307_220000/RConn3 -- T_79879307_220000_Sesto_San_Giovanni/LConn3 -- Brugherio_Sesto_CN_79879307_220000_CN_68299044_220000/LConn3 -- bus28/LConn1 -- _CN_79879290_220000_CN_79879307_220000/LConn3
  Sulcis_Oristano_CN_141046481_220000_CN_408799290_220000/LConn1 -- T_141046481_220000_Sottostazione_elettrica_Oristano/LConn1 -- Codrongianos_Oristano_CN_141046481_220000_CN_61743815_220000/LConn1
  Sulcis_Oristano_CN_141046481_220000_CN_408799290_220000/LConn2 -- T_141046481_220000_Sottostazione_elettrica_Oristano/LConn2 -- Codrongianos_Oristano_CN_141046481_220000_CN_61743815_220000/LConn2
  Sulcis_Oristano_CN_141046481_220000_CN_408799290_220000/LConn3 -- T_141046481_220000_Sottostazione_elettrica_Oristano/LConn3 -- Codrongianos_Oristano_CN_141046481_220000_CN_61743815_220000/LConn3 -- bus29/LConn1
  Sulcis_Oristano_CN_141046481_220000_CN_408799290_220000/RConn1 -- T_408799290_220000_Sulcis_Centrale/LConn1 -- Sulcis_Portoscuso_1_CN_408799290_220000_CN_375892276_220000/LConn1 -- Sulcis_Villasor_CN_408799290_220000_CN_144005861_220000/LConn1 -- Sulcis_Portoscuso_1_CN_408799290_220000_CN244933798/LConn1
  Sulcis_Oristano_CN_141046481_220000_CN_408799290_220000/RConn2 -- T_408799290_220000_Sulcis_Centrale/LConn2 -- Sulcis_Portoscuso_1_CN_408799290_220000_CN_375892276_220000/LConn2 -- Sulcis_Villasor_CN_408799290_220000_CN_144005861_220000/LConn2 -- Sulcis_Portoscuso_1_CN_408799290_220000_CN244933798/LConn2
  Sulcis_Oristano_CN_141046481_220000_CN_408799290_220000/RConn3 -- T_408799290_220000_Sulcis_Centrale/LConn3 -- Sulcis_Portoscuso_1_CN_408799290_220000_CN_375892276_220000/LConn3 -- bus30/LConn1 -- Sulcis_Villasor_CN_408799290_220000_CN_144005861_220000/LConn3 -- Sulcis_Portoscuso_1_CN_408799290_220000_CN244933798/LConn3
  Codrongianos_Oristano_CN_141046481_220000_CN_61743815_220000/RConn1 -- T_61743815_380000;220000;150000_Codrongianos/RConn1 -- Ottana_Codrongianos_CN_61743815_220000_CN_144006711_220000/LConn1
  Codrongianos_Oristano_CN_141046481_220000_CN_61743815_220000/RConn2 -- T_61743815_380000;220000;150000_Codrongianos/RConn2 -- Ottana_Codrongianos_CN_61743815_220000_CN_144006711_220000/LConn2
  Codrongianos_Oristano_CN_141046481_220000_CN_61743815_220000/RConn3 -- T_61743815_380000;220000;150000_Codrongianos/RConn3 -- Ottana_Codrongianos_CN_61743815_220000_CN_144006711_220000/LConn3 -- bus31/LConn1
  Villa_Castelli_Taranto_nord_CN_103381531_220000_CN_377300897_220000/LConn1 -- T_103381531_380000_Taranto_Nord/RConn4 -- _CN_103381531_220000_CN_185576620_220000/LConn1 -- Pisticci_Taranto_Nord_CN_103381531_220000_CN_104321356_220000/LConn1 -- _CN_103381531_220000_CN_185425637_220000/LConn1
  Villa_Castelli_Taranto_nord_CN_103381531_220000_CN_377300897_220000/LConn2 -- T_103381531_380000_Taranto_Nord/RConn5 -- _CN_103381531_220000_CN_185576620_220000/LConn2 -- Pisticci_Taranto_Nord_CN_103381531_220000_CN_104321356_220000/LConn2 -- _CN_103381531_220000_CN_185425637_220000/LConn2
  Villa_Castelli_Taranto_nord_CN_103381531_220000_CN_377300897_220000/LConn3 -- T_103381531_380000_Taranto_Nord/RConn6 -- _CN_103381531_220000_CN_185576620_220000/LConn3 -- Pisticci_Taranto_Nord_CN_103381531_220000_CN_104321356_220000/LConn3 -- _CN_103381531_220000_CN_185425637_220000/LConn3 -- bus32/LConn1
  Villa_Castelli_Taranto_nord_CN_103381531_220000_CN_377300897_220000/RConn1 -- T_377300897_220000_Villa_Castelli/LConn1 -- Villa_Castelli_Brindisi_CN_377300897_220000_CN_60919237_220000/LConn1
  Villa_Castelli_Taranto_nord_CN_103381531_220000_CN_377300897_220000/RConn2 -- T_377300897_220000_Villa_Castelli/LConn2 -- Villa_Castelli_Brindisi_CN_377300897_220000_CN_60919237_220000/LConn2
  Villa_Castelli_Taranto_nord_CN_103381531_220000_CN_377300897_220000/RConn3 -- T_377300897_220000_Villa_Castelli/LConn3 -- Villa_Castelli_Brindisi_CN_377300897_220000_CN_60919237_220000/LConn3 -- bus33/LConn1
  T_185576620_220000_/LConn1 -- _CN_103381531_220000_CN_185576620_220000/RConn1
  T_185576620_220000_/LConn2 -- _CN_103381531_220000_CN_185576620_220000/RConn2
  _CN_103381531_220000_CN_185576620_220000/RConn3 -- T_185576620_220000_/LConn3 -- bus34/LConn1
  Pisticci_Taranto_Nord_CN_103381531_220000_CN_104321356_220000/RConn1 -- T_104321356_220000_Pisticci/LConn1 -- Pisticci_Tecnoparco_CN_104321356_220000_CN_320030656_220000/LConn1
  Pisticci_Taranto_Nord_CN_103381531_220000_CN_104321356_220000/RConn2 -- T_104321356_220000_Pisticci/LConn2 -- Pisticci_Tecnoparco_CN_104321356_220000_CN_320030656_220000/LConn2
  Pisticci_Taranto_Nord_CN_103381531_220000_CN_104321356_220000/RConn3 -- T_104321356_220000_Pisticci/LConn3 -- Pisticci_Tecnoparco_CN_104321356_220000_CN_320030656_220000/LConn3 -- bus35/LConn1
  T_185425637__/LConn1 -- _CN_103381531_220000_CN_185425637_220000/RConn1
  T_185425637__/LConn2 -- _CN_103381531_220000_CN_185425637_220000/RConn2
  _CN_103381531_220000_CN_185425637_220000/RConn3 -- T_185425637__/LConn3 -- bus36/LConn1
  _CN_377830944_220000_CN_332123606_220000/LConn1 -- T_377830944_220000_Torino_Nord/LConn1 -- _CN_377830944_220000_CN_332123607_220000/LConn1
  _CN_377830944_220000_CN_332123606_220000/LConn2 -- T_377830944_220000_Torino_Nord/LConn2 -- _CN_377830944_220000_CN_332123607_220000/LConn2
  _CN_377830944_220000_CN_332123606_220000/LConn3 -- T_377830944_220000_Torino_Nord/LConn3 -- _CN_377830944_220000_CN_332123607_220000/LConn3 -- bus37/LConn1
  _CN_377830944_220000_CN_332123606_220000/RConn1 -- T_332123606__/LConn1 -- _CN_105153431_220000_CN_332123606_220000/LConn1
  _CN_377830944_220000_CN_332123606_220000/RConn2 -- T_332123606__/LConn2 -- _CN_105153431_220000_CN_332123606_220000/LConn2
  _CN_377830944_220000_CN_332123606_220000/RConn3 -- T_332123606__/LConn3 -- _CN_105153431_220000_CN_332123606_220000/LConn3 -- bus38/LConn1
  _CN_377830944_220000_CN_332123607_220000/RConn1 -- T_332123607__/LConn1 -- _CN_105062415_220000_CN_332123607_220000/LConn1
  _CN_377830944_220000_CN_332123607_220000/RConn2 -- T_332123607__/LConn2 -- _CN_105062415_220000_CN_332123607_220000/LConn2
  _CN_377830944_220000_CN_332123607_220000/RConn3 -- T_332123607__/LConn3 -- _CN_105062415_220000_CN_332123607_220000/LConn3 -- bus39/LConn1
  T_187150881_220000_Mucone_primo_salto/LConn1 -- Terranova_Mucone_secondo_salto_CN_187150881_220000_CN_187149304_220000/LConn1
  T_187150881_220000_Mucone_primo_salto/LConn2 -- Terranova_Mucone_secondo_salto_CN_187150881_220000_CN_187149304_220000/LConn2
  Terranova_Mucone_secondo_salto_CN_187150881_220000_CN_187149304_220000/LConn3 -- T_187150881_220000_Mucone_primo_salto/LConn3 -- bus40/LConn1
  Terranova_Mucone_secondo_salto_CN_187150881_220000_CN_187149304_220000/RConn1 -- T_187149304_220000_Terranova/LConn1 -- Rotonda_Terranova_CN_187149304_220000_CN_108020695_220000/LConn1
  Terranova_Mucone_secondo_salto_CN_187150881_220000_CN_187149304_220000/RConn2 -- T_187149304_220000_Terranova/LConn2 -- Rotonda_Terranova_CN_187149304_220000_CN_108020695_220000/LConn2
  Terranova_Mucone_secondo_salto_CN_187150881_220000_CN_187149304_220000/RConn3 -- T_187149304_220000_Terranova/LConn3 -- Rotonda_Terranova_CN_187149304_220000_CN_108020695_220000/LConn3 -- bus41/LConn1
  Casanova___Teksid_Carmagnola_CN_103974946_220000_CN_99826025_220000/LConn1 -- T_103974946_220000_Teksid_Carmagnola/LConn1 -- Casanova___Teksid_Carmagnola_CN_103974946_220000_CN_104239286_220000/LConn1 -- _CN_103974946_220000_CN_103525675_220000/LConn1
  Casanova___Teksid_Carmagnola_CN_103974946_220000_CN_99826025_220000/LConn2 -- T_103974946_220000_Teksid_Carmagnola/LConn2 -- Casanova___Teksid_Carmagnola_CN_103974946_220000_CN_104239286_220000/LConn2 -- _CN_103974946_220000_CN_103525675_220000/LConn2
  Casanova___Teksid_Carmagnola_CN_103974946_220000_CN_99826025_220000/LConn3 -- T_103974946_220000_Teksid_Carmagnola/LConn3 -- Casanova___Teksid_Carmagnola_CN_103974946_220000_CN_104239286_220000/LConn3 -- _CN_103974946_220000_CN_103525675_220000/LConn3 -- bus42/LConn1
  Casanova___Teksid_Carmagnola_CN_103974946_220000_CN_99826025_220000/RConn1 -- T_99826025_380000_Casanova/RConn4 -- Vignole_Borbera___Casanova_CN_99826025_220000_CN_100952845_220000/LConn1 -- _CN_99826025_220000_CN_103725268_220000/LConn1
  Casanova___Teksid_Carmagnola_CN_103974946_220000_CN_99826025_220000/RConn2 -- T_99826025_380000_Casanova/RConn5 -- Vignole_Borbera___Casanova_CN_99826025_220000_CN_100952845_220000/LConn2 -- _CN_99826025_220000_CN_103725268_220000/LConn2
  Casanova___Teksid_Carmagnola_CN_103974946_220000_CN_99826025_220000/RConn3 -- T_99826025_380000_Casanova/RConn6 -- Vignole_Borbera___Casanova_CN_99826025_220000_CN_100952845_220000/LConn3 -- bus43/LConn1 -- _CN_99826025_220000_CN_103725268_220000/LConn3
  Casanova___Teksid_Carmagnola_CN_103974946_220000_CN_104239286_220000/RConn1 -- T_104239286_220000_Bistagno/LConn1 -- Bistagno_Erzelli_CN_59629638_220000_CN_104239286_220000/LConn1
  Casanova___Teksid_Carmagnola_CN_103974946_220000_CN_104239286_220000/RConn2 -- T_104239286_220000_Bistagno/LConn2 -- Bistagno_Erzelli_CN_59629638_220000_CN_104239286_220000/LConn2
  Casanova___Teksid_Carmagnola_CN_103974946_220000_CN_104239286_220000/RConn3 -- T_104239286_220000_Bistagno/LConn3 -- Bistagno_Erzelli_CN_59629638_220000_CN_104239286_220000/LConn3 -- bus44/LConn1
  T_103525675_220000_Moncalieri_AEM/LConn1 -- _CN_103974946_220000_CN_103525675_220000/RConn1
  T_103525675_220000_Moncalieri_AEM/LConn2 -- _CN_103974946_220000_CN_103525675_220000/RConn2
  _CN_103974946_220000_CN_103525675_220000/RConn3 -- T_103525675_220000_Moncalieri_AEM/LConn3 -- bus45/LConn1
  T_108050523_220000;132000_FS_Nomentana/LConn1 -- _CN_108050523_220000_CN_80517630_220000/LConn1
  T_108050523_220000;132000_FS_Nomentana/LConn2 -- _CN_108050523_220000_CN_80517630_220000/LConn2
  _CN_108050523_220000_CN_80517630_220000/LConn3 -- T_108050523_220000;132000_FS_Nomentana/LConn3 -- bus46/LConn1
  _CN_108050523_220000_CN_80517630_220000/RConn1 -- T_80517630_380000_Roma_Nord_smistamento_energia_elettrica_TERNA/RConn4 -- SantaLucia_Roma_Nord_CN_84963374_220000_CN_80517630_220000/LConn1 -- SantaLucia_Roma_Nord_2_CN_165371026_220000_CN_80517630_220000/LConn1
  _CN_108050523_220000_CN_80517630_220000/RConn2 -- T_80517630_380000_Roma_Nord_smistamento_energia_elettrica_TERNA/RConn5 -- SantaLucia_Roma_Nord_CN_84963374_220000_CN_80517630_220000/LConn2 -- SantaLucia_Roma_Nord_2_CN_165371026_220000_CN_80517630_220000/LConn2
  _CN_108050523_220000_CN_80517630_220000/RConn3 -- T_80517630_380000_Roma_Nord_smistamento_energia_elettrica_TERNA/RConn6 -- SantaLucia_Roma_Nord_CN_84963374_220000_CN_80517630_220000/LConn3 -- SantaLucia_Roma_Nord_2_CN_165371026_220000_CN_80517630_220000/LConn3 -- bus47/LConn1
  T_173659686_220000_Enichem_Ottana/LConn1 -- _CN_173659686_220000_CN_144006711_220000/LConn1
  T_173659686_220000_Enichem_Ottana/LConn2 -- _CN_173659686_220000_CN_144006711_220000/LConn2
  _CN_173659686_220000_CN_144006711_220000/LConn3 -- T_173659686_220000_Enichem_Ottana/LConn3 -- bus48/LConn1
  _CN_173659686_220000_CN_144006711_220000/RConn1 -- T_144006711_220000_Ottana/LConn1 -- Ottana_Busachi_CN_210352180_220000_CN_144006711_220000/LConn1 -- Ottana_Taloro_1_CN_144006711_220000_CN139974542/LConn1 -- Ottana_Codrongianos_CN_61743815_220000_CN_144006711_220000/RConn1
  _CN_173659686_220000_CN_144006711_220000/RConn2 -- T_144006711_220000_Ottana/LConn2 -- Ottana_Busachi_CN_210352180_220000_CN_144006711_220000/LConn2 -- Ottana_Taloro_1_CN_144006711_220000_CN139974542/LConn2 -- Ottana_Codrongianos_CN_61743815_220000_CN_144006711_220000/RConn2
  _CN_173659686_220000_CN_144006711_220000/RConn3 -- T_144006711_220000_Ottana/LConn3 -- Ottana_Busachi_CN_210352180_220000_CN_144006711_220000/LConn3 -- Ottana_Taloro_1_CN_144006711_220000_CN139974542/LConn3 -- bus49/LConn1 -- Ottana_Codrongianos_CN_61743815_220000_CN_144006711_220000/RConn3
  T_41360305_380000_Poggio_a_Caiano/RConn4 -- _CN_41360305_220000_CN_139975773_220000/LConn1
  T_41360305_380000_Poggio_a_Caiano/RConn5 -- _CN_41360305_220000_CN_139975773_220000/LConn2
  _CN_41360305_220000_CN_139975773_220000/LConn3 -- T_41360305_380000_Poggio_a_Caiano/RConn6 -- bus50/LConn1
  T_139975773_380000_Casellina/RConn4 -- _CN_41360305_220000_CN_139975773_220000/RConn1
  T_139975773_380000_Casellina/RConn5 -- _CN_41360305_220000_CN_139975773_220000/RConn2
  _CN_41360305_220000_CN_139975773_220000/RConn3 -- T_139975773_380000_Casellina/RConn6 -- bus51/LConn1
  Patria_San_Antimo_CN_132455976_220000_CN_114661587_220000/RConn1 -- T_132455976_220000_Sant'Antimo/LConn1 -- Fratta_San_Antimo_CN_132455976_220000_CN_132702940_220000/LConn1 -- Patria_San_Antimo_CN_132455976_220000_CN_132725149_220000/LConn1
  Patria_San_Antimo_CN_132455976_220000_CN_114661587_220000/RConn2 -- T_132455976_220000_Sant'Antimo/LConn2 -- Fratta_San_Antimo_CN_132455976_220000_CN_132702940_220000/LConn2 -- Patria_San_Antimo_CN_132455976_220000_CN_132725149_220000/LConn2
  Patria_San_Antimo_CN_132455976_220000_CN_114661587_220000/RConn3 -- T_132455976_220000_Sant'Antimo/LConn3 -- Fratta_San_Antimo_CN_132455976_220000_CN_132702940_220000/LConn3 -- bus52/LConn1 -- Patria_San_Antimo_CN_132455976_220000_CN_132725149_220000/LConn3
  Patria_San_Antimo_CN_132455976_220000_CN_132725149_220000/RConn1 -- T_132725149_220000_Astroni/LConn1 -- Astroni_Arenella_CN_132725149_220000_CN_377588144_220000/LConn1 -- Astroni_Patria_CN_114661587_220000_CN_132725149_220000/RConn1 -- Astroni_Pozzuoli_CN_132726160_220000_CN_132725149_220000/LConn1
  Patria_San_Antimo_CN_132455976_220000_CN_132725149_220000/RConn2 -- T_132725149_220000_Astroni/LConn2 -- Astroni_Arenella_CN_132725149_220000_CN_377588144_220000/LConn2 -- Astroni_Patria_CN_114661587_220000_CN_132725149_220000/RConn2 -- Astroni_Pozzuoli_CN_132726160_220000_CN_132725149_220000/LConn2
  Patria_San_Antimo_CN_132455976_220000_CN_132725149_220000/RConn3 -- T_132725149_220000_Astroni/LConn3 -- Astroni_Arenella_CN_132725149_220000_CN_377588144_220000/LConn3 -- bus53/LConn1 -- Astroni_Patria_CN_114661587_220000_CN_132725149_220000/RConn3 -- Astroni_Pozzuoli_CN_132726160_220000_CN_132725149_220000/LConn3
  Fratta_San_Antimo_CN_132455976_220000_CN_132702940_220000/RConn1 -- T_132702940_60000;220000_Frattamaggiore/LConn1 -- Fratta_Poggioreale_CN_93850768_220000_CN_132702940_220000/LConn1 -- Aversa_Fratta_CN_132701980_220000_CN_132702940_220000/LConn1 -- Fratta_Maddaloni_CN_132702940_220000_CN_132717802_220000/LConn1 -- Fratta_Maddaloni_CN_132702940_220000_CN_377588184_220000/LConn1 -- Casalnuovo_Fratta_CN_132702940_220000_CN_370679021_220000/LConn1 -- Acerra_Fratta_CN_132702940_220000_CN_132701023_220000/LConn1
  Fratta_San_Antimo_CN_132455976_220000_CN_132702940_220000/RConn2 -- T_132702940_60000;220000_Frattamaggiore/LConn2 -- Fratta_Poggioreale_CN_93850768_220000_CN_132702940_220000/LConn2 -- Aversa_Fratta_CN_132701980_220000_CN_132702940_220000/LConn2 -- Fratta_Maddaloni_CN_132702940_220000_CN_132717802_220000/LConn2 -- Fratta_Maddaloni_CN_132702940_220000_CN_377588184_220000/LConn2 -- Casalnuovo_Fratta_CN_132702940_220000_CN_370679021_220000/LConn2 -- Acerra_Fratta_CN_132702940_220000_CN_132701023_220000/LConn2
  Fratta_San_Antimo_CN_132455976_220000_CN_132702940_220000/RConn3 -- T_132702940_60000;220000_Frattamaggiore/LConn3 -- Fratta_Poggioreale_CN_93850768_220000_CN_132702940_220000/LConn3 -- Aversa_Fratta_CN_132701980_220000_CN_132702940_220000/LConn3 -- Fratta_Maddaloni_CN_132702940_220000_CN_132717802_220000/LConn3 -- Fratta_Maddaloni_CN_132702940_220000_CN_377588184_220000/LConn3 -- Casalnuovo_Fratta_CN_132702940_220000_CN_370679021_220000/LConn3 -- Acerra_Fratta_CN_132702940_220000_CN_132701023_220000/LConn3 -- bus54/LConn1
  Montorio_Candia_CN_36873258_220000_CN_136457747_220000/LConn1 -- T_36873258_380000_Candia/RConn4 -- Montorio_Candia_CN_36873258_220000_CN_158652469_220000/LConn1
  Montorio_Candia_CN_36873258_220000_CN_136457747_220000/LConn2 -- T_36873258_380000_Candia/RConn5 -- Montorio_Candia_CN_36873258_220000_CN_158652469_220000/LConn2
  Montorio_Candia_CN_36873258_220000_CN_136457747_220000/LConn3 -- T_36873258_380000_Candia/RConn6 -- Montorio_Candia_CN_36873258_220000_CN_158652469_220000/LConn3 -- bus55/LConn1
  T_136457747_220000_Abbadia/LConn1 -- Montorio_Candia_CN_36873258_220000_CN_136457747_220000/RConn1
  T_136457747_220000_Abbadia/LConn2 -- Montorio_Candia_CN_36873258_220000_CN_136457747_220000/RConn2
  Montorio_Candia_CN_36873258_220000_CN_136457747_220000/RConn3 -- T_136457747_220000_Abbadia/LConn3 -- bus56/LConn1
  Montorio_Candia_CN_36873258_220000_CN_158652469_220000/RConn1 -- T_158652469_220000_Montorio/LConn1 -- Montorio_Villanova_CN_61375111_220000_CN_158652469_220000/LConn1
  Montorio_Candia_CN_36873258_220000_CN_158652469_220000/RConn2 -- T_158652469_220000_Montorio/LConn2 -- Montorio_Villanova_CN_61375111_220000_CN_158652469_220000/LConn2
  Montorio_Candia_CN_36873258_220000_CN_158652469_220000/RConn3 -- T_158652469_220000_Montorio/LConn3 -- Montorio_Villanova_CN_61375111_220000_CN_158652469_220000/LConn3 -- bus57/LConn1
  Scorzè___Soverzene_CN_159821869_220000_CN_128602121_220000/LConn1 -- T_159821869_220000_Soverzene/LConn1 -- Scorzè___Soverzene_CN_159821869_220000_CN111346267/LConn1 -- Fadalto___Soverzene_CN_159821869_220000_CN_155976582_220000/LConn1
  Scorzè___Soverzene_CN_159821869_220000_CN_128602121_220000/LConn2 -- T_159821869_220000_Soverzene/LConn2 -- Scorzè___Soverzene_CN_159821869_220000_CN111346267/LConn2 -- Fadalto___Soverzene_CN_159821869_220000_CN_155976582_220000/LConn2
  Scorzè___Soverzene_CN_159821869_220000_CN_128602121_220000/LConn3 -- T_159821869_220000_Soverzene/LConn3 -- Scorzè___Soverzene_CN_159821869_220000_CN111346267/LConn3 -- Fadalto___Soverzene_CN_159821869_220000_CN_155976582_220000/LConn3 -- bus58/LConn1
  Scorzè___Soverzene_CN_159821869_220000_CN_128602121_220000/RConn1 -- T_128602121_220000_Scorzè/LConn1 -- Scorzè___Treviso_Sud_CN_128602121_220000_CN_59026315_220000/LConn1 -- _CN_128602121_220000_CN_59366523_220000/LConn1 -- Scorzè_Malcontenta_CN_128602121_220000_CN_281091768_220000/LConn1 -- Scorzè_Malcontenta_CN_128602121_220000_CN_202272734_220000/LConn1 -- Scorzè_Dolo_CN_128602121_220000_CN_59153311_220000/LConn1
  Scorzè___Soverzene_CN_159821869_220000_CN_128602121_220000/RConn2 -- T_128602121_220000_Scorzè/LConn2 -- Scorzè___Treviso_Sud_CN_128602121_220000_CN_59026315_220000/LConn2 -- _CN_128602121_220000_CN_59366523_220000/LConn2 -- Scorzè_Malcontenta_CN_128602121_220000_CN_281091768_220000/LConn2 -- Scorzè_Malcontenta_CN_128602121_220000_CN_202272734_220000/LConn2 -- Scorzè_Dolo_CN_128602121_220000_CN_59153311_220000/LConn2
  Scorzè___Soverzene_CN_159821869_220000_CN_128602121_220000/RConn3 -- T_128602121_220000_Scorzè/LConn3 -- Scorzè___Treviso_Sud_CN_128602121_220000_CN_59026315_220000/LConn3 -- _CN_128602121_220000_CN_59366523_220000/LConn3 -- bus59/LConn1 -- Scorzè_Malcontenta_CN_128602121_220000_CN_281091768_220000/LConn3 -- Scorzè_Malcontenta_CN_128602121_220000_CN_202272734_220000/LConn3 -- Scorzè_Dolo_CN_128602121_220000_CN_59153311_220000/LConn3
  "G_111346267_Centrale_idroelettrica_\"Achille_Gaggia\""/RConn1 -- Scorzè___Soverzene_CN_159821869_220000_CN111346267/RConn1
  "G_111346267_Centrale_idroelettrica_\"Achille_Gaggia\""/RConn2 -- Scorzè___Soverzene_CN_159821869_220000_CN111346267/RConn2
  Scorzè___Soverzene_CN_159821869_220000_CN111346267/RConn3 -- "G_111346267_Centrale_idroelettrica_\"Achille_Gaggia\""/RConn3 -- bus60/LConn1
  Fadalto___Soverzene_CN_159821869_220000_CN_155976582_220000/RConn1 -- T_155976582_220000_Fadalto/LConn1 -- _CN_155976563_220000_CN_155976582_220000/LConn1
  Fadalto___Soverzene_CN_159821869_220000_CN_155976582_220000/RConn2 -- T_155976582_220000_Fadalto/LConn2 -- _CN_155976563_220000_CN_155976582_220000/LConn2
  Fadalto___Soverzene_CN_159821869_220000_CN_155976582_220000/RConn3 -- T_155976582_220000_Fadalto/LConn3 -- _CN_155976563_220000_CN_155976582_220000/LConn3 -- bus61/LConn1
  SantaLucia_Roma_Nord_CN_84963374_220000_CN_165371026_220000/LConn1 -- T_84963374_220000_Flaminia/LConn1 -- SantaLucia_Roma_Nord_CN_84963374_220000_CN_80517630_220000/RConn1
  SantaLucia_Roma_Nord_CN_84963374_220000_CN_165371026_220000/LConn2 -- T_84963374_220000_Flaminia/LConn2 -- SantaLucia_Roma_Nord_CN_84963374_220000_CN_80517630_220000/RConn2
  SantaLucia_Roma_Nord_CN_84963374_220000_CN_165371026_220000/LConn3 -- T_84963374_220000_Flaminia/LConn3 -- SantaLucia_Roma_Nord_CN_84963374_220000_CN_80517630_220000/RConn3 -- bus62/LConn1
  SantaLucia_Roma_Nord_CN_84963374_220000_CN_165371026_220000/RConn1 -- T_165371026__/LConn1 -- SantaLucia_Roma_Nord_2_CN_165371026_220000_CN_80517630_220000/RConn1 -- _CN_165371026_220000_CN_165371027_220000/LConn1
  SantaLucia_Roma_Nord_CN_84963374_220000_CN_165371026_220000/RConn2 -- T_165371026__/LConn2 -- SantaLucia_Roma_Nord_2_CN_165371026_220000_CN_80517630_220000/RConn2 -- _CN_165371026_220000_CN_165371027_220000/LConn2
  SantaLucia_Roma_Nord_CN_84963374_220000_CN_165371026_220000/RConn3 -- T_165371026__/LConn3 -- SantaLucia_Roma_Nord_2_CN_165371026_220000_CN_80517630_220000/RConn3 -- bus63/LConn1 -- _CN_165371026_220000_CN_165371027_220000/LConn3
  Lana_Sant'Antonio_CN_42862642_220000_CN_105827045_220000/RConn1 -- T_105827045_220000_Sant'Antonio/LConn1 -- _CN_105827045_220000_CN_105801489_220000/LConn1
  Lana_Sant'Antonio_CN_42862642_220000_CN_105827045_220000/RConn2 -- T_105827045_220000_Sant'Antonio/LConn2 -- _CN_105827045_220000_CN_105801489_220000/LConn2
  Lana_Sant'Antonio_CN_42862642_220000_CN_105827045_220000/RConn3 -- T_105827045_220000_Sant'Antonio/LConn3 -- _CN_105827045_220000_CN_105801489_220000/LConn3 -- bus64/LConn1
  Lana_Sant'Antonio_CN_42862642_220000_CN_105801489_220000/RConn1 -- T_105801489_220000_Kardaun___Cardano/LConn1 -- _CN_105827045_220000_CN_105801489_220000/RConn1
  Lana_Sant'Antonio_CN_42862642_220000_CN_105801489_220000/RConn2 -- T_105801489_220000_Kardaun___Cardano/LConn2 -- _CN_105827045_220000_CN_105801489_220000/RConn2
  Lana_Sant'Antonio_CN_42862642_220000_CN_105801489_220000/RConn3 -- T_105801489_220000_Kardaun___Cardano/LConn3 -- _CN_105827045_220000_CN_105801489_220000/RConn3 -- bus65/LConn1
  Lana_Sant'Antonio_CN_42862642_220000_CN_147466201_220000/RConn1 -- T_147466201_220000_Santa_Massenza_Centrale/LConn1 -- _CN_147453809_220000_CN_147466201_220000/LConn1 -- Cimego_Santa_Massenza_CN_147466201_220000_CN_82793962_220000/LConn1 -- Lavis_Trento_sud_CN_96658563_220000_CN_147466201_220000/LConn1 -- Santa_Massenza_Bussolengo_CN_111020792_220000_CN_147466201_220000/LConn1 -- Gargnano_Nave_CN_189137043_220000_CN_147466201_220000/LConn1 -- Taio_Santa_Massenza_CN_147455038_220000_CN_147466201_220000/LConn1
  Lana_Sant'Antonio_CN_42862642_220000_CN_147466201_220000/RConn2 -- T_147466201_220000_Santa_Massenza_Centrale/LConn2 -- _CN_147453809_220000_CN_147466201_220000/LConn2 -- Cimego_Santa_Massenza_CN_147466201_220000_CN_82793962_220000/LConn2 -- Lavis_Trento_sud_CN_96658563_220000_CN_147466201_220000/LConn2 -- Santa_Massenza_Bussolengo_CN_111020792_220000_CN_147466201_220000/LConn2 -- Gargnano_Nave_CN_189137043_220000_CN_147466201_220000/LConn2 -- Taio_Santa_Massenza_CN_147455038_220000_CN_147466201_220000/LConn2
  Lana_Sant'Antonio_CN_42862642_220000_CN_147466201_220000/RConn3 -- T_147466201_220000_Santa_Massenza_Centrale/LConn3 -- _CN_147453809_220000_CN_147466201_220000/LConn3 -- Cimego_Santa_Massenza_CN_147466201_220000_CN_82793962_220000/LConn3 -- bus66/LConn1 -- Lavis_Trento_sud_CN_96658563_220000_CN_147466201_220000/LConn3 -- Santa_Massenza_Bussolengo_CN_111020792_220000_CN_147466201_220000/LConn3 -- Gargnano_Nave_CN_189137043_220000_CN_147466201_220000/LConn3 -- Taio_Santa_Massenza_CN_147455038_220000_CN_147466201_220000/LConn3
  _CN_166196787_220000_CN_75378894_220000/LConn1 -- T_166196787_220000_Dalmine_BG/LConn1 -- derivazione_Dalmine_CN_166196787_220000_CN_68299044_220000/LConn1
  _CN_166196787_220000_CN_75378894_220000/LConn2 -- T_166196787_220000_Dalmine_BG/LConn2 -- derivazione_Dalmine_CN_166196787_220000_CN_68299044_220000/LConn2
  _CN_166196787_220000_CN_75378894_220000/LConn3 -- T_166196787_220000_Dalmine_BG/LConn3 -- derivazione_Dalmine_CN_166196787_220000_CN_68299044_220000/LConn3 -- bus67/LConn1
  _CN_166196787_220000_CN_75378894_220000/RConn1 -- T_75378894_380000_Cislago/RConn4 -- _CN_163056522_220000_CN_75378894_220000/LConn1
  _CN_166196787_220000_CN_75378894_220000/RConn2 -- T_75378894_380000_Cislago/RConn5 -- _CN_163056522_220000_CN_75378894_220000/LConn2
  _CN_166196787_220000_CN_75378894_220000/RConn3 -- T_75378894_380000_Cislago/RConn6 -- _CN_163056522_220000_CN_75378894_220000/LConn3 -- bus68/LConn1
  derivazione_Dalmine_CN_166196787_220000_CN_68299044_220000/RConn1 -- T_68299044_380000_Brugherio___Smistamento_elettrico_TERNA/RConn4 -- _CN_163958919_220000_CN_68299044_220000/LConn1 -- _CN_79879290_220000_CN_68299044_220000/LConn1 -- Brugherio_Sesto_CN_79879307_220000_CN_68299044_220000/RConn1
  derivazione_Dalmine_CN_166196787_220000_CN_68299044_220000/RConn2 -- T_68299044_380000_Brugherio___Smistamento_elettrico_TERNA/RConn5 -- _CN_163958919_220000_CN_68299044_220000/LConn2 -- _CN_79879290_220000_CN_68299044_220000/LConn2 -- Brugherio_Sesto_CN_79879307_220000_CN_68299044_220000/RConn2
  derivazione_Dalmine_CN_166196787_220000_CN_68299044_220000/RConn3 -- T_68299044_380000_Brugherio___Smistamento_elettrico_TERNA/RConn6 -- _CN_163958919_220000_CN_68299044_220000/LConn3 -- _CN_79879290_220000_CN_68299044_220000/LConn3 -- Brugherio_Sesto_CN_79879307_220000_CN_68299044_220000/RConn3 -- bus69/LConn1
  Novara_Sud_Magenta_CN_103264820_220000_CN_67461115_220000/LConn1 -- T_103264820_220000_Magenta/LConn1 -- Baggio_Magenta_CN_103264820_220000_CN_62326314_220000/LConn1 -- _CN_103264820_220000_CN_104114052_220000/LConn1
  Novara_Sud_Magenta_CN_103264820_220000_CN_67461115_220000/LConn2 -- T_103264820_220000_Magenta/LConn2 -- Baggio_Magenta_CN_103264820_220000_CN_62326314_220000/LConn2 -- _CN_103264820_220000_CN_104114052_220000/LConn2
  Novara_Sud_Magenta_CN_103264820_220000_CN_67461115_220000/LConn3 -- T_103264820_220000_Magenta/LConn3 -- Baggio_Magenta_CN_103264820_220000_CN_62326314_220000/LConn3 -- _CN_103264820_220000_CN_104114052_220000/LConn3 -- bus70/LConn1
  Novara_Sud_Magenta_CN_103264820_220000_CN_67461115_220000/RConn1 -- T_67461115_220000_Novara_Sud/LConn1 -- Vercelli_Novara_Sud_CN_98638424_220000_CN_67461115_220000/RConn1
  Novara_Sud_Magenta_CN_103264820_220000_CN_67461115_220000/RConn2 -- T_67461115_220000_Novara_Sud/LConn2 -- Vercelli_Novara_Sud_CN_98638424_220000_CN_67461115_220000/RConn2
  Novara_Sud_Magenta_CN_103264820_220000_CN_67461115_220000/RConn3 -- T_67461115_220000_Novara_Sud/LConn3 -- Vercelli_Novara_Sud_CN_98638424_220000_CN_67461115_220000/RConn3 -- bus71/LConn1
  Baggio_Magenta_CN_103264820_220000_CN_62326314_220000/RConn1 -- T_62326314_380000_Baggio/RConn4 -- _CN_62326314_220000_CN_136708548_220000/LConn1
  Baggio_Magenta_CN_103264820_220000_CN_62326314_220000/RConn2 -- T_62326314_380000_Baggio/RConn5 -- _CN_62326314_220000_CN_136708548_220000/LConn2
  Baggio_Magenta_CN_103264820_220000_CN_62326314_220000/RConn3 -- T_62326314_380000_Baggio/RConn6 -- _CN_62326314_220000_CN_136708548_220000/LConn3 -- bus72/LConn1
  _CN_103264820_220000_CN_104114052_220000/RConn1 -- T_104114052_220000_Pallanzeno_1/LConn1 -- Pallanzeno_Verampio_CN_103418587_220000_CN_104114052_220000/RConn1
  _CN_103264820_220000_CN_104114052_220000/RConn2 -- T_104114052_220000_Pallanzeno_1/LConn2 -- Pallanzeno_Verampio_CN_103418587_220000_CN_104114052_220000/RConn2
  _CN_103264820_220000_CN_104114052_220000/RConn3 -- T_104114052_220000_Pallanzeno_1/LConn3 -- Pallanzeno_Verampio_CN_103418587_220000_CN_104114052_220000/RConn3 -- bus73/LConn1
  Cassano_Brescia_Ricevitrice_Ovest_CN_133601333_220000_CN_116692433_220000/LConn1 -- T_133601333_220000_Cassano_220/LConn1 -- _CN_133601333_220000_CN_135270825_220000/LConn1 -- Milano_Ricevitrice_Nord_Cassano_CN_133601333_220000_CN67400512/LConn1
  Cassano_Brescia_Ricevitrice_Ovest_CN_133601333_220000_CN_116692433_220000/LConn2 -- T_133601333_220000_Cassano_220/LConn2 -- _CN_133601333_220000_CN_135270825_220000/LConn2 -- Milano_Ricevitrice_Nord_Cassano_CN_133601333_220000_CN67400512/LConn2
  Cassano_Brescia_Ricevitrice_Ovest_CN_133601333_220000_CN_116692433_220000/LConn3 -- T_133601333_220000_Cassano_220/LConn3 -- _CN_133601333_220000_CN_135270825_220000/LConn3 -- Milano_Ricevitrice_Nord_Cassano_CN_133601333_220000_CN67400512/LConn3 -- bus74/LConn1
  T_116692433_220000_Brescia_Ricevitrice_Ovest/LConn1 -- Cassano_Brescia_Ricevitrice_Ovest_CN_133601333_220000_CN_116692433_220000/RConn1
  T_116692433_220000_Brescia_Ricevitrice_Ovest/LConn2 -- Cassano_Brescia_Ricevitrice_Ovest_CN_133601333_220000_CN_116692433_220000/RConn2
  Cassano_Brescia_Ricevitrice_Ovest_CN_133601333_220000_CN_116692433_220000/RConn3 -- T_116692433_220000_Brescia_Ricevitrice_Ovest/LConn3 -- bus75/LConn1
  _CN_133601333_220000_CN_135270825_220000/RConn1 -- T_135270825_220000_Ricevitrice_Sud_Milano/LConn1 -- Grosio_Milano_Ricevitrice_Sud_CN_80442466_220000_CN_135270825_220000/LConn1 -- Milano_Ricevitrice_Sud_Tavazzano_CN_116916459_220000_CN_135270825_220000/LConn1
  _CN_133601333_220000_CN_135270825_220000/RConn2 -- T_135270825_220000_Ricevitrice_Sud_Milano/LConn2 -- Grosio_Milano_Ricevitrice_Sud_CN_80442466_220000_CN_135270825_220000/LConn2 -- Milano_Ricevitrice_Sud_Tavazzano_CN_116916459_220000_CN_135270825_220000/LConn2
  _CN_133601333_220000_CN_135270825_220000/RConn3 -- T_135270825_220000_Ricevitrice_Sud_Milano/LConn3 -- Grosio_Milano_Ricevitrice_Sud_CN_80442466_220000_CN_135270825_220000/LConn3 -- Milano_Ricevitrice_Sud_Tavazzano_CN_116916459_220000_CN_135270825_220000/LConn3 -- bus76/LConn1
  Milano_Ricevitrice_Nord_Cassano_CN_133601333_220000_CN67400512/RConn1 -- G_67400512_Centrale_di_Cassano_d'Adda/RConn1 -- _CN_79879290_220000_CN67400512/LConn1
  Milano_Ricevitrice_Nord_Cassano_CN_133601333_220000_CN67400512/RConn2 -- G_67400512_Centrale_di_Cassano_d'Adda/RConn2 -- _CN_79879290_220000_CN67400512/LConn2
  Milano_Ricevitrice_Nord_Cassano_CN_133601333_220000_CN67400512/RConn3 -- G_67400512_Centrale_di_Cassano_d'Adda/RConn3 -- _CN_79879290_220000_CN67400512/LConn3 -- bus77/LConn1
  Scorzè_Malcontenta_CN_128602121_220000_CN_281091768_220000/RConn1 -- T_281091768__Malcontenta/LConn1 -- _CN_281091768_220000_CN_129406824_220000/LConn1 -- _CN_281091768_220000_CN_129407370_220000/LConn1 -- _CN_281091768_220000_CN_59153311_220000/LConn1 -- _CN_281091768_220000_CN_416679117_220000/LConn1
  Scorzè_Malcontenta_CN_128602121_220000_CN_281091768_220000/RConn2 -- T_281091768__Malcontenta/LConn2 -- _CN_281091768_220000_CN_129406824_220000/LConn2 -- _CN_281091768_220000_CN_129407370_220000/LConn2 -- _CN_281091768_220000_CN_59153311_220000/LConn2 -- _CN_281091768_220000_CN_416679117_220000/LConn2
  Scorzè_Malcontenta_CN_128602121_220000_CN_281091768_220000/RConn3 -- T_281091768__Malcontenta/LConn3 -- _CN_281091768_220000_CN_129406824_220000/LConn3 -- bus78/LConn1 -- _CN_281091768_220000_CN_129407370_220000/LConn3 -- _CN_281091768_220000_CN_59153311_220000/LConn3 -- _CN_281091768_220000_CN_416679117_220000/LConn3
  Scorzè_Malcontenta_CN_128602121_220000_CN_202272734_220000/RConn1 -- T_202272734_220000_Castegnero/LConn1 -- Sandrà_Dugale_CN_156001963_220000_CN_202272734_220000/LConn1 -- Castegnero___Cittadella_CN_149188707_220000_CN_202272734_220000/LConn1
  Scorzè_Malcontenta_CN_128602121_220000_CN_202272734_220000/RConn2 -- T_202272734_220000_Castegnero/LConn2 -- Sandrà_Dugale_CN_156001963_220000_CN_202272734_220000/LConn2 -- Castegnero___Cittadella_CN_149188707_220000_CN_202272734_220000/LConn2
  Scorzè_Malcontenta_CN_128602121_220000_CN_202272734_220000/RConn3 -- T_202272734_220000_Castegnero/LConn3 -- Sandrà_Dugale_CN_156001963_220000_CN_202272734_220000/LConn3 -- bus79/LConn1 -- Castegnero___Cittadella_CN_149188707_220000_CN_202272734_220000/LConn3
  Scorzè_Dolo_CN_128602121_220000_CN_59153311_220000/RConn1 -- T_59153311_380000_Dolo/RConn4 -- Dolo___Fusina_CN_100407576_220000_CN_59153311_220000/LConn1 -- Camin___Dolo_CN_59366523_220000_CN_59153311_220000/LConn1 -- _CN_281091768_220000_CN_59153311_220000/RConn1
  Scorzè_Dolo_CN_128602121_220000_CN_59153311_220000/RConn2 -- T_59153311_380000_Dolo/RConn5 -- Dolo___Fusina_CN_100407576_220000_CN_59153311_220000/LConn2 -- Camin___Dolo_CN_59366523_220000_CN_59153311_220000/LConn2 -- _CN_281091768_220000_CN_59153311_220000/RConn2
  Scorzè_Dolo_CN_128602121_220000_CN_59153311_220000/RConn3 -- T_59153311_380000_Dolo/RConn6 -- Dolo___Fusina_CN_100407576_220000_CN_59153311_220000/LConn3 -- bus80/LConn1 -- Camin___Dolo_CN_59366523_220000_CN_59153311_220000/LConn3 -- _CN_281091768_220000_CN_59153311_220000/RConn3
  Scorzè___Treviso_Sud_CN_128602121_220000_CN_59026315_220000/RConn1 -- T_59026315_380000_Salgareda/RConn4 -- Somplago_Pordenone_CN_61650514_220000_CN_59026315_220000/LConn1 -- _CN_155976563_220000_CN_59026315_220000/LConn1
  Scorzè___Treviso_Sud_CN_128602121_220000_CN_59026315_220000/RConn2 -- T_59026315_380000_Salgareda/RConn5 -- Somplago_Pordenone_CN_61650514_220000_CN_59026315_220000/LConn2 -- _CN_155976563_220000_CN_59026315_220000/LConn2
  Scorzè___Treviso_Sud_CN_128602121_220000_CN_59026315_220000/RConn3 -- T_59026315_380000_Salgareda/RConn6 -- Somplago_Pordenone_CN_61650514_220000_CN_59026315_220000/LConn3 -- _CN_155976563_220000_CN_59026315_220000/LConn3 -- bus81/LConn1
  _CN_128602121_220000_CN_59366523_220000/RConn1 -- T_59366523_380000;220000;132000_Stazione_elettrica_di_Camin/RConn1 -- Camin___Dolo_CN_59366523_220000_CN_59153311_220000/RConn1 -- Camin_Acciaierie_Venete_CN_128523865_220000_CN_59366523_220000/LConn1
  _CN_128602121_220000_CN_59366523_220000/RConn2 -- T_59366523_380000;220000;132000_Stazione_elettrica_di_Camin/RConn2 -- Camin___Dolo_CN_59366523_220000_CN_59153311_220000/RConn2 -- Camin_Acciaierie_Venete_CN_128523865_220000_CN_59366523_220000/LConn2
  _CN_128602121_220000_CN_59366523_220000/RConn3 -- T_59366523_380000;220000;132000_Stazione_elettrica_di_Camin/RConn3 -- Camin___Dolo_CN_59366523_220000_CN_59153311_220000/RConn3 -- bus82/LConn1 -- Camin_Acciaierie_Venete_CN_128523865_220000_CN_59366523_220000/LConn3
  Sulcis_Villasor_CN_408799290_220000_CN_144005861_220000/RConn1 -- T_144005861_220000_Villasor_Centrale/LConn1 -- Selargius_Villasor_CN_118987056_220000_CN_144005861_220000/LConn1 -- Mogorella_Villasor_CN_210352188_220000_CN_144005861_220000/LConn1
  Sulcis_Villasor_CN_408799290_220000_CN_144005861_220000/RConn2 -- T_144005861_220000_Villasor_Centrale/LConn2 -- Selargius_Villasor_CN_118987056_220000_CN_144005861_220000/LConn2 -- Mogorella_Villasor_CN_210352188_220000_CN_144005861_220000/LConn2
  Sulcis_Villasor_CN_408799290_220000_CN_144005861_220000/RConn3 -- T_144005861_220000_Villasor_Centrale/LConn3 -- Selargius_Villasor_CN_118987056_220000_CN_144005861_220000/LConn3 -- bus83/LConn1 -- Mogorella_Villasor_CN_210352188_220000_CN_144005861_220000/LConn3
  "G_244933798_Centrale_termoelettrica_\"Grazia_Deledda\""/RConn1 -- Sulcis_Portoscuso_1_CN_408799290_220000_CN244933798/RConn1
  "G_244933798_Centrale_termoelettrica_\"Grazia_Deledda\""/RConn2 -- Sulcis_Portoscuso_1_CN_408799290_220000_CN244933798/RConn2
  Sulcis_Portoscuso_1_CN_408799290_220000_CN244933798/RConn3 -- "G_244933798_Centrale_termoelettrica_\"Grazia_Deledda\""/RConn3 -- bus84/LConn1
  T_375892276_220000_Portoscuso/LConn1 -- Sulcis_Portoscuso_1_CN_408799290_220000_CN_375892276_220000/RConn1
  T_375892276_220000_Portoscuso/LConn2 -- Sulcis_Portoscuso_1_CN_408799290_220000_CN_375892276_220000/RConn2
  Sulcis_Portoscuso_1_CN_408799290_220000_CN_375892276_220000/RConn3 -- T_375892276_220000_Portoscuso/LConn3 -- bus85/LConn1
  _CN_57384507_220000_CN_57380344_220000/LConn1 -- T_57384507_380000_Chiaramonte_Gulfi/RConn4 -- _CN_57384507_220000_CN_56984450_220000/LConn1
  _CN_57384507_220000_CN_57380344_220000/LConn2 -- T_57384507_380000_Chiaramonte_Gulfi/RConn5 -- _CN_57384507_220000_CN_56984450_220000/LConn2
  _CN_57384507_220000_CN_57380344_220000/LConn3 -- T_57384507_380000_Chiaramonte_Gulfi/RConn6 -- _CN_57384507_220000_CN_56984450_220000/LConn3 -- bus86/LConn1
  _CN_57384507_220000_CN_57380344_220000/RConn1 -- T_57380344_220000_Ragusa/LConn1 -- Ragusa_Polimeri_Europa_CN_375922075_220000_CN_57380344_220000/LConn1
  _CN_57384507_220000_CN_57380344_220000/RConn2 -- T_57380344_220000_Ragusa/LConn2 -- Ragusa_Polimeri_Europa_CN_375922075_220000_CN_57380344_220000/LConn2
  _CN_57384507_220000_CN_57380344_220000/RConn3 -- T_57380344_220000_Ragusa/LConn3 -- Ragusa_Polimeri_Europa_CN_375922075_220000_CN_57380344_220000/LConn3 -- bus87/LConn1
  _CN_57384507_220000_CN_56984450_220000/RConn1 -- T_56984450_220000_Favara/LConn1 -- _CN_375916035_220000_CN_56984450_220000/LConn1
  _CN_57384507_220000_CN_56984450_220000/RConn2 -- T_56984450_220000_Favara/LConn2 -- _CN_375916035_220000_CN_56984450_220000/LConn2
  _CN_57384507_220000_CN_56984450_220000/RConn3 -- T_56984450_220000_Favara/LConn3 -- _CN_375916035_220000_CN_56984450_220000/LConn3 -- bus88/LConn1
  Mogorella_Busachi_CN_210352188_220000_CN_210352180_220000/LConn1 -- T_210352188_220000_Ghrighine_Centrale/LConn1 -- Mogorella_Villasor_CN_210352188_220000_CN_144005861_220000/RConn1
  Mogorella_Busachi_CN_210352188_220000_CN_210352180_220000/LConn2 -- T_210352188_220000_Ghrighine_Centrale/LConn2 -- Mogorella_Villasor_CN_210352188_220000_CN_144005861_220000/RConn2
  Mogorella_Busachi_CN_210352188_220000_CN_210352180_220000/LConn3 -- T_210352188_220000_Ghrighine_Centrale/LConn3 -- Mogorella_Villasor_CN_210352188_220000_CN_144005861_220000/RConn3 -- bus89/LConn1
  Mogorella_Busachi_CN_210352188_220000_CN_210352180_220000/RConn1 -- T_210352180_220000_CenTrale_Tirso/LConn1 -- Ottana_Busachi_CN_210352180_220000_CN_144006711_220000/RConn1
  Mogorella_Busachi_CN_210352188_220000_CN_210352180_220000/RConn2 -- T_210352180_220000_CenTrale_Tirso/LConn2 -- Ottana_Busachi_CN_210352180_220000_CN_144006711_220000/RConn2
  Mogorella_Busachi_CN_210352188_220000_CN_210352180_220000/RConn3 -- T_210352180_220000_CenTrale_Tirso/LConn3 -- Ottana_Busachi_CN_210352180_220000_CN_144006711_220000/RConn3 -- bus90/LConn1
  Salerno_Nord_Montecorvino_CN_85196861_220000_CN_376952616_220000/LConn1 -- T_85196861_380000_Montecorvino/RConn4 -- _CN_85196861_220000_CN_85297730_220000/LConn1 -- Montecorvino_Tusciano_CN_85196861_220000_CN_420698910_220000/LConn1 -- Salerno_Nord_Montecorvino_CN_85196861_220000_CN_124220303_220000/LConn1
  Salerno_Nord_Montecorvino_CN_85196861_220000_CN_376952616_220000/LConn2 -- T_85196861_380000_Montecorvino/RConn5 -- _CN_85196861_220000_CN_85297730_220000/LConn2 -- Montecorvino_Tusciano_CN_85196861_220000_CN_420698910_220000/LConn2 -- Salerno_Nord_Montecorvino_CN_85196861_220000_CN_124220303_220000/LConn2
  Salerno_Nord_Montecorvino_CN_85196861_220000_CN_376952616_220000/LConn3 -- T_85196861_380000_Montecorvino/RConn6 -- _CN_85196861_220000_CN_85297730_220000/LConn3 -- bus91/LConn1 -- Montecorvino_Tusciano_CN_85196861_220000_CN_420698910_220000/LConn3 -- Salerno_Nord_Montecorvino_CN_85196861_220000_CN_124220303_220000/LConn3
  Salerno_Nord_Montecorvino_CN_85196861_220000_CN_376952616_220000/RConn1 -- T_376952616_220000_Nocera/LConn1 -- Nola_San_Valentino_CN_202711181_220000_CN_376952616_220000/LConn1
  Salerno_Nord_Montecorvino_CN_85196861_220000_CN_376952616_220000/RConn2 -- T_376952616_220000_Nocera/LConn2 -- Nola_San_Valentino_CN_202711181_220000_CN_376952616_220000/LConn2
  Salerno_Nord_Montecorvino_CN_85196861_220000_CN_376952616_220000/RConn3 -- T_376952616_220000_Nocera/LConn3 -- Nola_San_Valentino_CN_202711181_220000_CN_376952616_220000/LConn3 -- bus92/LConn1
  T_124220303_220000_Salerno_Nord/LConn1 -- Salerno_Nord_Montecorvino_CN_85196861_220000_CN_124220303_220000/RConn1
  T_124220303_220000_Salerno_Nord/LConn2 -- Salerno_Nord_Montecorvino_CN_85196861_220000_CN_124220303_220000/RConn2
  Salerno_Nord_Montecorvino_CN_85196861_220000_CN_124220303_220000/RConn3 -- T_124220303_220000_Salerno_Nord/LConn3 -- bus93/LConn1
  Montecorvino_Tusciano_CN_85196861_220000_CN_420698910_220000/RConn1 -- T_420698910_220000_Tusciano/LConn1 -- Rotonda_Tusciano_CN_420698910_220000_CN_108020695_220000/LConn1
  Montecorvino_Tusciano_CN_85196861_220000_CN_420698910_220000/RConn2 -- T_420698910_220000_Tusciano/LConn2 -- Rotonda_Tusciano_CN_420698910_220000_CN_108020695_220000/LConn2
  Montecorvino_Tusciano_CN_85196861_220000_CN_420698910_220000/RConn3 -- T_420698910_220000_Tusciano/LConn3 -- Rotonda_Tusciano_CN_420698910_220000_CN_108020695_220000/LConn3 -- bus94/LConn1
  _CN_85196861_220000_CN_85297730_220000/RConn1 -- T_85297730_220000_Gragnano/LConn1 -- Gragnano_Torre_Nord_CN_85297730_220000_CN_114659171_220000/LConn1
  _CN_85196861_220000_CN_85297730_220000/RConn2 -- T_85297730_220000_Gragnano/LConn2 -- Gragnano_Torre_Nord_CN_85297730_220000_CN_114659171_220000/LConn2
  _CN_85196861_220000_CN_85297730_220000/RConn3 -- T_85297730_220000_Gragnano/LConn3 -- Gragnano_Torre_Nord_CN_85297730_220000_CN_114659171_220000/LConn3 -- bus95/LConn1
  Taio_Santa_Massenza_CN_147455038_220000_CN96654904/LConn1 -- T_147455038_220000_Santa_Massenza_Smistamento/LConn1 -- Taio_Santa_Massenza_CN_147455038_220000_CN_156001963_220000/LConn1 -- Taio_Santa_Massenza_CN_147455038_220000_CN_147466201_220000/RConn1
  Taio_Santa_Massenza_CN_147455038_220000_CN96654904/LConn2 -- T_147455038_220000_Santa_Massenza_Smistamento/LConn2 -- Taio_Santa_Massenza_CN_147455038_220000_CN_156001963_220000/LConn2 -- Taio_Santa_Massenza_CN_147455038_220000_CN_147466201_220000/RConn2
  Taio_Santa_Massenza_CN_147455038_220000_CN96654904/LConn3 -- T_147455038_220000_Santa_Massenza_Smistamento/LConn3 -- Taio_Santa_Massenza_CN_147455038_220000_CN_156001963_220000/LConn3 -- Taio_Santa_Massenza_CN_147455038_220000_CN_147466201_220000/RConn3 -- bus96/LConn1
  Taio_Santa_Massenza_CN_147455038_220000_CN96654904/RConn1 -- G_96654904_/RConn1 -- Taio_Cedegolo_CN_281837810_220000_CN96654904/LConn1
  Taio_Santa_Massenza_CN_147455038_220000_CN96654904/RConn2 -- G_96654904_/RConn2 -- Taio_Cedegolo_CN_281837810_220000_CN96654904/LConn2
  Taio_Santa_Massenza_CN_147455038_220000_CN96654904/RConn3 -- G_96654904_/RConn3 -- Taio_Cedegolo_CN_281837810_220000_CN96654904/LConn3 -- bus97/LConn1
  Taio_Santa_Massenza_CN_147455038_220000_CN_156001963_220000/RConn1 -- T_156001963_220000_Stazione_elettrica_di_Sandrà/LConn1 -- Sandrà_Colà_CN_156001963_220000_CN_156001981_220000/LConn1 -- Sandrà_Bussolengo_CN_156001963_220000_CN_111020792_220000/LConn1 -- Sandrà_Dugale_CN_156001963_220000_CN_59556712_220000/LConn1 -- Sandrà_Dugale_CN_156001963_220000_CN_202272734_220000/RConn1 -- Sandrà_Mantova_CN_156001963_220000_CN_412909650_220000/LConn1
  Taio_Santa_Massenza_CN_147455038_220000_CN_156001963_220000/RConn2 -- T_156001963_220000_Stazione_elettrica_di_Sandrà/LConn2 -- Sandrà_Colà_CN_156001963_220000_CN_156001981_220000/LConn2 -- Sandrà_Bussolengo_CN_156001963_220000_CN_111020792_220000/LConn2 -- Sandrà_Dugale_CN_156001963_220000_CN_59556712_220000/LConn2 -- Sandrà_Dugale_CN_156001963_220000_CN_202272734_220000/RConn2 -- Sandrà_Mantova_CN_156001963_220000_CN_412909650_220000/LConn2
  Taio_Santa_Massenza_CN_147455038_220000_CN_156001963_220000/RConn3 -- T_156001963_220000_Stazione_elettrica_di_Sandrà/LConn3 -- Sandrà_Colà_CN_156001963_220000_CN_156001981_220000/LConn3 -- bus98/LConn1 -- Sandrà_Bussolengo_CN_156001963_220000_CN_111020792_220000/LConn3 -- Sandrà_Dugale_CN_156001963_220000_CN_59556712_220000/LConn3 -- Sandrà_Dugale_CN_156001963_220000_CN_202272734_220000/RConn3 -- Sandrà_Mantova_CN_156001963_220000_CN_412909650_220000/LConn3
  Brusciano_Nola_CN_132638645_220000_CN_202711181_220000/LConn1 -- T_132638645_220000_Brusciano/LConn1 -- Fiat_Auto_Brusciano_CN_132638645_220000_CN_132637884_220000/LConn1 -- Brusciano_Alfa_Avio_CN_132638645_220000_CN_132638412_220000/LConn1 -- Brusciano_Maddaloni_CN_132638645_220000_CN_132701023_220000/LConn1 -- Brusciano_Maddaloni_CN_132638645_220000_CN_132717802_220000/LConn1
  Brusciano_Nola_CN_132638645_220000_CN_202711181_220000/LConn2 -- T_132638645_220000_Brusciano/LConn2 -- Fiat_Auto_Brusciano_CN_132638645_220000_CN_132637884_220000/LConn2 -- Brusciano_Alfa_Avio_CN_132638645_220000_CN_132638412_220000/LConn2 -- Brusciano_Maddaloni_CN_132638645_220000_CN_132701023_220000/LConn2 -- Brusciano_Maddaloni_CN_132638645_220000_CN_132717802_220000/LConn2
  Brusciano_Nola_CN_132638645_220000_CN_202711181_220000/LConn3 -- T_132638645_220000_Brusciano/LConn3 -- Fiat_Auto_Brusciano_CN_132638645_220000_CN_132637884_220000/LConn3 -- Brusciano_Alfa_Avio_CN_132638645_220000_CN_132638412_220000/LConn3 -- Brusciano_Maddaloni_CN_132638645_220000_CN_132701023_220000/LConn3 -- Brusciano_Maddaloni_CN_132638645_220000_CN_132717802_220000/LConn3 -- bus99/LConn1
  Brusciano_Nola_CN_132638645_220000_CN_202711181_220000/RConn1 -- T_202711181_220000_Nola/LConn1 -- Nola_San_Valentino_CN_202711181_220000_CN_376952616_220000/RConn1
  Brusciano_Nola_CN_132638645_220000_CN_202711181_220000/RConn2 -- T_202711181_220000_Nola/LConn2 -- Nola_San_Valentino_CN_202711181_220000_CN_376952616_220000/RConn2
  Brusciano_Nola_CN_132638645_220000_CN_202711181_220000/RConn3 -- T_202711181_220000_Nola/LConn3 -- Nola_San_Valentino_CN_202711181_220000_CN_376952616_220000/RConn3 -- bus100/LConn1
  Fiat_Auto_Brusciano_CN_132638645_220000_CN_132637884_220000/RConn1 -- T_132637884_220000_Fiat_Auto/LConn1 -- Fiat_Auto_Maddaloni_CN_132637884_220000_CN_132717802_220000/LConn1
  Fiat_Auto_Brusciano_CN_132638645_220000_CN_132637884_220000/RConn2 -- T_132637884_220000_Fiat_Auto/LConn2 -- Fiat_Auto_Maddaloni_CN_132637884_220000_CN_132717802_220000/LConn2
  Fiat_Auto_Brusciano_CN_132638645_220000_CN_132637884_220000/RConn3 -- T_132637884_220000_Fiat_Auto/LConn3 -- Fiat_Auto_Maddaloni_CN_132637884_220000_CN_132717802_220000/LConn3 -- bus101/LConn1
  Brusciano_Alfa_Avio_CN_132638645_220000_CN_132638412_220000/RConn1 -- T_132638412__/LConn1 -- _CN_132638412_220000_CN_376952600_220000/LConn1
  Brusciano_Alfa_Avio_CN_132638645_220000_CN_132638412_220000/RConn2 -- T_132638412__/LConn2 -- _CN_132638412_220000_CN_376952600_220000/LConn2
  Brusciano_Alfa_Avio_CN_132638645_220000_CN_132638412_220000/RConn3 -- T_132638412__/LConn3 -- _CN_132638412_220000_CN_376952600_220000/LConn3 -- bus102/LConn1
  Brusciano_Maddaloni_CN_132638645_220000_CN_132701023_220000/RConn1 -- T_132701023_220000_Acerra_smistamento/LConn1 -- Acerra_Fratta_CN_132702940_220000_CN_132701023_220000/RConn1
  Brusciano_Maddaloni_CN_132638645_220000_CN_132701023_220000/RConn2 -- T_132701023_220000_Acerra_smistamento/LConn2 -- Acerra_Fratta_CN_132702940_220000_CN_132701023_220000/RConn2
  Brusciano_Maddaloni_CN_132638645_220000_CN_132701023_220000/RConn3 -- T_132701023_220000_Acerra_smistamento/LConn3 -- Acerra_Fratta_CN_132702940_220000_CN_132701023_220000/RConn3 -- bus103/LConn1
  Brusciano_Maddaloni_CN_132638645_220000_CN_132717802_220000/RConn1 -- T_132717802_220000_Maddaloni/LConn1 -- Fiat_Auto_Maddaloni_CN_132637884_220000_CN_132717802_220000/RConn1 -- Fratta_Maddaloni_CN_132702940_220000_CN_132717802_220000/RConn1 -- Maddaloni_Air_Liquide_CN_132719324_220000_CN_132717802_220000/LConn1 -- Maddaloni_Santa_Sofia_CN_132717802_220000_CN_84696559_220000/LConn1
  Brusciano_Maddaloni_CN_132638645_220000_CN_132717802_220000/RConn2 -- T_132717802_220000_Maddaloni/LConn2 -- Fiat_Auto_Maddaloni_CN_132637884_220000_CN_132717802_220000/RConn2 -- Fratta_Maddaloni_CN_132702940_220000_CN_132717802_220000/RConn2 -- Maddaloni_Air_Liquide_CN_132719324_220000_CN_132717802_220000/LConn2 -- Maddaloni_Santa_Sofia_CN_132717802_220000_CN_84696559_220000/LConn2
  Brusciano_Maddaloni_CN_132638645_220000_CN_132717802_220000/RConn3 -- T_132717802_220000_Maddaloni/LConn3 -- Fiat_Auto_Maddaloni_CN_132637884_220000_CN_132717802_220000/RConn3 -- Fratta_Maddaloni_CN_132702940_220000_CN_132717802_220000/RConn3 -- Maddaloni_Air_Liquide_CN_132719324_220000_CN_132717802_220000/LConn3 -- Maddaloni_Santa_Sofia_CN_132717802_220000_CN_84696559_220000/LConn3 -- bus104/LConn1
  Belviso_Venina_CN_163789376_220000_CN163056519/LConn1 -- T_163789376_220000_Venina/LConn1 -- Venina_Cassano_CS_CN_163789376_220000_CN_75947658_220000/LConn1
  Belviso_Venina_CN_163789376_220000_CN163056519/LConn2 -- T_163789376_220000_Venina/LConn2 -- Venina_Cassano_CS_CN_163789376_220000_CN_75947658_220000/LConn2
  Belviso_Venina_CN_163789376_220000_CN163056519/LConn3 -- T_163789376_220000_Venina/LConn3 -- Venina_Cassano_CS_CN_163789376_220000_CN_75947658_220000/LConn3 -- bus105/LConn1
  Belviso_Venina_CN_163789376_220000_CN163056519/RConn1 -- G_163056519_Centrale_di_Belviso/RConn1 -- Belviso_Ganda_CN_202772821_220000_CN163056519/LConn1
  Belviso_Venina_CN_163789376_220000_CN163056519/RConn2 -- G_163056519_Centrale_di_Belviso/RConn2 -- Belviso_Ganda_CN_202772821_220000_CN163056519/LConn2
  Belviso_Venina_CN_163789376_220000_CN163056519/RConn3 -- G_163056519_Centrale_di_Belviso/RConn3 -- Belviso_Ganda_CN_202772821_220000_CN163056519/LConn3 -- bus106/LConn1
  Venina_Cassano_CS_CN_163789376_220000_CN_75947658_220000/RConn1 -- T_75947658_220000_Cassano_CS/LConn1 -- Cassano_Tavazzano_Ovest_CN_75947658_220000_CN_107241327_220000/LConn1 -- _CN_75947658_220000_CN_203468251_220000/LConn1
  Venina_Cassano_CS_CN_163789376_220000_CN_75947658_220000/RConn2 -- T_75947658_220000_Cassano_CS/LConn2 -- Cassano_Tavazzano_Ovest_CN_75947658_220000_CN_107241327_220000/LConn2 -- _CN_75947658_220000_CN_203468251_220000/LConn2
  Venina_Cassano_CS_CN_163789376_220000_CN_75947658_220000/RConn3 -- T_75947658_220000_Cassano_CS/LConn3 -- Cassano_Tavazzano_Ovest_CN_75947658_220000_CN_107241327_220000/LConn3 -- _CN_75947658_220000_CN_203468251_220000/LConn3 -- bus107/LConn1
  T_114659171_220000_/LConn1 -- Gragnano_Torre_Nord_CN_85297730_220000_CN_114659171_220000/RConn1
  T_114659171_220000_/LConn2 -- Gragnano_Torre_Nord_CN_85297730_220000_CN_114659171_220000/RConn2
  Gragnano_Torre_Nord_CN_85297730_220000_CN_114659171_220000/RConn3 -- T_114659171_220000_/LConn3 -- bus108/LConn1
  Lanzada_Sondrio_CN_318173253_220000_CN_163056526_220000/LConn1 -- T_318173253__/LConn1 -- Lanzada_Sondrio_CN_318173253_220000_CN_163056522_220000/LConn1
  Lanzada_Sondrio_CN_318173253_220000_CN_163056526_220000/LConn2 -- T_318173253__/LConn2 -- Lanzada_Sondrio_CN_318173253_220000_CN_163056522_220000/LConn2
  Lanzada_Sondrio_CN_318173253_220000_CN_163056526_220000/LConn3 -- T_318173253__/LConn3 -- Lanzada_Sondrio_CN_318173253_220000_CN_163056522_220000/LConn3 -- bus109/LConn1
  Lanzada_Sondrio_CN_318173253_220000_CN_163056526_220000/RConn1 -- T_163056526_220000_Lanzada/LConn1 -- Lanzada_Campo_Moro_CN_348500306_220000_CN_163056526_220000/LConn1
  Lanzada_Sondrio_CN_318173253_220000_CN_163056526_220000/RConn2 -- T_163056526_220000_Lanzada/LConn2 -- Lanzada_Campo_Moro_CN_348500306_220000_CN_163056526_220000/LConn2
  Lanzada_Sondrio_CN_318173253_220000_CN_163056526_220000/RConn3 -- T_163056526_220000_Lanzada/LConn3 -- Lanzada_Campo_Moro_CN_348500306_220000_CN_163056526_220000/LConn3 -- bus110/LConn1
  Lanzada_Sondrio_CN_318173253_220000_CN_163056522_220000/RConn1 -- T_163056522_220000_Sondrio/LConn1 -- _CN_163056522_220000_CN_75378894_220000/RConn1
  Lanzada_Sondrio_CN_318173253_220000_CN_163056522_220000/RConn2 -- T_163056522_220000_Sondrio/LConn2 -- _CN_163056522_220000_CN_75378894_220000/RConn2
  Lanzada_Sondrio_CN_318173253_220000_CN_163056522_220000/RConn3 -- T_163056522_220000_Sondrio/LConn3 -- _CN_163056522_220000_CN_75378894_220000/RConn3 -- bus111/LConn1
  Bistagno_Erzelli_CN_59629638_220000_CN_104239286_220000/RConn1 -- T_59629638_220000_Erzelli/LConn1 -- Erzelli_Morigallo_CN_59629638_220000_CN_61484190_220000/LConn1
  Bistagno_Erzelli_CN_59629638_220000_CN_104239286_220000/RConn2 -- T_59629638_220000_Erzelli/LConn2 -- Erzelli_Morigallo_CN_59629638_220000_CN_61484190_220000/LConn2
  Bistagno_Erzelli_CN_59629638_220000_CN_104239286_220000/RConn3 -- T_59629638_220000_Erzelli/LConn3 -- Erzelli_Morigallo_CN_59629638_220000_CN_61484190_220000/LConn3 -- bus112/LConn1
  Erzelli_Morigallo_CN_59629638_220000_CN_61484190_220000/RConn1 -- T_61484190_220000_Morigallo/LConn1 -- Morigallo_Savona_CN_61484190_220000_CN_296141722_220000/LConn1 -- Morigallo_Vignole_CN_61484190_220000_CN_100952845_220000/LConn1 -- Morigallo_San_Colombano_Certenoli_CN_61484190_220000_CN_103653565_220000/LConn1 -- Morigallo_San_Colombano_Certenoli_CN_61484190_220000_CN_158599954_220000/LConn1
  Erzelli_Morigallo_CN_59629638_220000_CN_61484190_220000/RConn2 -- T_61484190_220000_Morigallo/LConn2 -- Morigallo_Savona_CN_61484190_220000_CN_296141722_220000/LConn2 -- Morigallo_Vignole_CN_61484190_220000_CN_100952845_220000/LConn2 -- Morigallo_San_Colombano_Certenoli_CN_61484190_220000_CN_103653565_220000/LConn2 -- Morigallo_San_Colombano_Certenoli_CN_61484190_220000_CN_158599954_220000/LConn2
  Erzelli_Morigallo_CN_59629638_220000_CN_61484190_220000/RConn3 -- T_61484190_220000_Morigallo/LConn3 -- Morigallo_Savona_CN_61484190_220000_CN_296141722_220000/LConn3 -- Morigallo_Vignole_CN_61484190_220000_CN_100952845_220000/LConn3 -- bus113/LConn1 -- Morigallo_San_Colombano_Certenoli_CN_61484190_220000_CN_103653565_220000/LConn3 -- Morigallo_San_Colombano_Certenoli_CN_61484190_220000_CN_158599954_220000/LConn3
  Casalnuovo_Alfa_Avio_CN_376952589_220000_CN_370679021_220000/LConn1 -- T_376952589_220000_/LConn1 -- _CN_376952589_220000_CN_376952600_220000/LConn1
  Casalnuovo_Alfa_Avio_CN_376952589_220000_CN_370679021_220000/LConn2 -- T_376952589_220000_/LConn2 -- _CN_376952589_220000_CN_376952600_220000/LConn2
  Casalnuovo_Alfa_Avio_CN_376952589_220000_CN_370679021_220000/LConn3 -- T_376952589_220000_/LConn3 -- _CN_376952589_220000_CN_376952600_220000/LConn3 -- bus114/LConn1
  Casalnuovo_Alfa_Avio_CN_376952589_220000_CN_370679021_220000/RConn1 -- T_370679021_220000_Casalnuovo/LConn1 -- Casalnuovo_Fratta_CN_132702940_220000_CN_370679021_220000/RConn1 -- Castelluccia_Casalnuovo_CN_93850768_220000_CN_370679021_220000/LConn1
  Casalnuovo_Alfa_Avio_CN_376952589_220000_CN_370679021_220000/RConn2 -- T_370679021_220000_Casalnuovo/LConn2 -- Casalnuovo_Fratta_CN_132702940_220000_CN_370679021_220000/RConn2 -- Castelluccia_Casalnuovo_CN_93850768_220000_CN_370679021_220000/LConn2
  Casalnuovo_Alfa_Avio_CN_376952589_220000_CN_370679021_220000/RConn3 -- T_370679021_220000_Casalnuovo/LConn3 -- Casalnuovo_Fratta_CN_132702940_220000_CN_370679021_220000/RConn3 -- bus115/LConn1 -- Castelluccia_Casalnuovo_CN_93850768_220000_CN_370679021_220000/LConn3
  _CN_376952589_220000_CN_376952600_220000/RConn1 -- T_376952600_220000_Alfa_Avio/LConn1 -- _CN_132638412_220000_CN_376952600_220000/RConn1
  _CN_376952589_220000_CN_376952600_220000/RConn2 -- T_376952600_220000_Alfa_Avio/LConn2 -- _CN_132638412_220000_CN_376952600_220000/RConn2
  _CN_376952589_220000_CN_376952600_220000/RConn3 -- T_376952600_220000_Alfa_Avio/LConn3 -- _CN_132638412_220000_CN_376952600_220000/RConn3 -- bus116/LConn1
  T_199886416_220000_Mercure/LConn1 -- Mercure_Rotonda_CN_199886416_220000_CN_108020695_220000/LConn1
  T_199886416_220000_Mercure/LConn2 -- Mercure_Rotonda_CN_199886416_220000_CN_108020695_220000/LConn2
  Mercure_Rotonda_CN_199886416_220000_CN_108020695_220000/LConn3 -- T_199886416_220000_Mercure/LConn3 -- bus117/LConn1
  Mercure_Rotonda_CN_199886416_220000_CN_108020695_220000/RConn1 -- T_108020695_220000_Rotonda/LConn1 -- Laino_Rotonda_CN_108020416_220000_CN_108020695_220000/LConn1 -- Rotonda_Tusciano_CN_420698910_220000_CN_108020695_220000/RConn1 -- Rotonda_Terranova_CN_187149304_220000_CN_108020695_220000/RConn1
  Mercure_Rotonda_CN_199886416_220000_CN_108020695_220000/RConn2 -- T_108020695_220000_Rotonda/LConn2 -- Laino_Rotonda_CN_108020416_220000_CN_108020695_220000/LConn2 -- Rotonda_Tusciano_CN_420698910_220000_CN_108020695_220000/RConn2 -- Rotonda_Terranova_CN_187149304_220000_CN_108020695_220000/RConn2
  Mercure_Rotonda_CN_199886416_220000_CN_108020695_220000/RConn3 -- T_108020695_220000_Rotonda/LConn3 -- Laino_Rotonda_CN_108020416_220000_CN_108020695_220000/LConn3 -- Rotonda_Tusciano_CN_420698910_220000_CN_108020695_220000/RConn3 -- Rotonda_Terranova_CN_187149304_220000_CN_108020695_220000/RConn3 -- bus118/LConn1
  T_129407370_220000_Stazione_IV/LConn1 -- _CN_281091768_220000_CN_129407370_220000/RConn1
  T_129407370_220000_Stazione_IV/LConn2 -- _CN_281091768_220000_CN_129407370_220000/RConn2
  _CN_281091768_220000_CN_129407370_220000/RConn3 -- T_129407370_220000_Stazione_IV/LConn3 -- bus119/LConn1
  T_416679117_220000_Villabona/LConn1 -- _CN_281091768_220000_CN_416679117_220000/RConn1
  T_416679117_220000_Villabona/LConn2 -- _CN_281091768_220000_CN_416679117_220000/RConn2
  _CN_281091768_220000_CN_416679117_220000/RConn3 -- T_416679117_220000_Villabona/LConn3 -- bus120/LConn1
  T_129406824_220000;132000_Azotati/LConn1 -- _CN_281091768_220000_CN_129406824_220000/RConn1
  T_129406824_220000;132000_Azotati/LConn2 -- _CN_281091768_220000_CN_129406824_220000/RConn2
  _CN_281091768_220000_CN_129406824_220000/RConn3 -- T_129406824_220000;132000_Azotati/LConn3 -- bus121/LConn1
  T_61650514_220000_Somplago_centrale/LConn1 -- Somplago_Pordenone_CN_61650514_220000_CN_59026315_220000/RConn1
  T_61650514_220000_Somplago_centrale/LConn2 -- Somplago_Pordenone_CN_61650514_220000_CN_59026315_220000/RConn2
  Somplago_Pordenone_CN_61650514_220000_CN_59026315_220000/RConn3 -- T_61650514_220000_Somplago_centrale/LConn3 -- bus122/LConn1
  T_149188707_220000_Cittadella/LConn1 -- Castegnero___Cittadella_CN_149188707_220000_CN_202272734_220000/RConn1
  T_149188707_220000_Cittadella/LConn2 -- Castegnero___Cittadella_CN_149188707_220000_CN_202272734_220000/RConn2
  Castegnero___Cittadella_CN_149188707_220000_CN_202272734_220000/RConn3 -- T_149188707_220000_Cittadella/LConn3 -- bus123/LConn1
  T_128523865_220000_Acciaierie_Venete_220/LConn1 -- Camin_Acciaierie_Venete_CN_128523865_220000_CN_59366523_220000/RConn1
  T_128523865_220000_Acciaierie_Venete_220/LConn2 -- Camin_Acciaierie_Venete_CN_128523865_220000_CN_59366523_220000/RConn2
  Camin_Acciaierie_Venete_CN_128523865_220000_CN_59366523_220000/RConn3 -- T_128523865_220000_Acciaierie_Venete_220/LConn3 -- bus124/LConn1
  Martinetto_Pianezza_CN_105062415_220000_CN_58516664_220000/LConn1 -- T_105062415_220000_Pianezza/LConn1 -- Pianezza_Piossasco_CN_105062415_220000_CN_98902899_220000/LConn1 -- _CN_105062415_220000_CN_105141350_220000/LConn1 -- _CN_105062415_220000_CN_66872608_220000/LConn1 -- _CN_105062415_220000_CN_332123607_220000/RConn1
  Martinetto_Pianezza_CN_105062415_220000_CN_58516664_220000/LConn2 -- T_105062415_220000_Pianezza/LConn2 -- Pianezza_Piossasco_CN_105062415_220000_CN_98902899_220000/LConn2 -- _CN_105062415_220000_CN_105141350_220000/LConn2 -- _CN_105062415_220000_CN_66872608_220000/LConn2 -- _CN_105062415_220000_CN_332123607_220000/RConn2
  Martinetto_Pianezza_CN_105062415_220000_CN_58516664_220000/LConn3 -- T_105062415_220000_Pianezza/LConn3 -- Pianezza_Piossasco_CN_105062415_220000_CN_98902899_220000/LConn3 -- bus125/LConn1 -- _CN_105062415_220000_CN_105141350_220000/LConn3 -- _CN_105062415_220000_CN_66872608_220000/LConn3 -- _CN_105062415_220000_CN_332123607_220000/RConn3
  T_58516664_220000_Martinetto/LConn1 -- Martinetto_Pianezza_CN_105062415_220000_CN_58516664_220000/RConn1
  T_58516664_220000_Martinetto/LConn2 -- Martinetto_Pianezza_CN_105062415_220000_CN_58516664_220000/RConn2
  Martinetto_Pianezza_CN_105062415_220000_CN_58516664_220000/RConn3 -- T_58516664_220000_Martinetto/LConn3 -- bus126/LConn1
  T_105141350_220000_Grugliasco/LConn1 -- _CN_105062415_220000_CN_105141350_220000/RConn1
  T_105141350_220000_Grugliasco/LConn2 -- _CN_105062415_220000_CN_105141350_220000/RConn2
  _CN_105062415_220000_CN_105141350_220000/RConn3 -- T_105141350_220000_Grugliasco/LConn3 -- bus127/LConn1
  _CN_105062415_220000_CN_66872608_220000/RConn1 -- T_66872608_220000_Rosone/LConn1 -- Villa___Rosone_CN_66872608_220000_CN_102185356_220000/LConn1
  _CN_105062415_220000_CN_66872608_220000/RConn2 -- T_66872608_220000_Rosone/LConn2 -- Villa___Rosone_CN_66872608_220000_CN_102185356_220000/LConn2
  _CN_105062415_220000_CN_66872608_220000/RConn3 -- T_66872608_220000_Rosone/LConn3 -- Villa___Rosone_CN_66872608_220000_CN_102185356_220000/LConn3 -- bus128/LConn1
  T_98902899_380000_Piossasco/RConn4 -- Pianezza_Piossasco_CN_105062415_220000_CN_98902899_220000/RConn1
  T_98902899_380000_Piossasco/RConn5 -- Pianezza_Piossasco_CN_105062415_220000_CN_98902899_220000/RConn2
  Pianezza_Piossasco_CN_105062415_220000_CN_98902899_220000/RConn3 -- T_98902899_380000_Piossasco/RConn6 -- bus129/LConn1
  Lambrate_Cesi_CN_163958919_220000_CN_203771704_220000/LConn1 -- T_163958919_220000_Lambrate/LConn1 -- _CN_163958919_220000_CN_68299044_220000/RConn1
  Lambrate_Cesi_CN_163958919_220000_CN_203771704_220000/LConn2 -- T_163958919_220000_Lambrate/LConn2 -- _CN_163958919_220000_CN_68299044_220000/RConn2
  Lambrate_Cesi_CN_163958919_220000_CN_203771704_220000/LConn3 -- T_163958919_220000_Lambrate/LConn3 -- _CN_163958919_220000_CN_68299044_220000/RConn3 -- bus130/LConn1
  T_203771704_220000_UT_CESI/LConn1 -- Lambrate_Cesi_CN_163958919_220000_CN_203771704_220000/RConn1
  T_203771704_220000_UT_CESI/LConn2 -- Lambrate_Cesi_CN_163958919_220000_CN_203771704_220000/RConn2
  Lambrate_Cesi_CN_163958919_220000_CN_203771704_220000/RConn3 -- T_203771704_220000_UT_CESI/LConn3 -- bus131/LConn1
  _CN_173999201_220000_CN_376502734_220000/LConn1 -- T_173999201_220000_Napoli_Levante/LConn1 -- _CN_173999201_220000_CN_377444648_220000/LConn1
  _CN_173999201_220000_CN_376502734_220000/LConn2 -- T_173999201_220000_Napoli_Levante/LConn2 -- _CN_173999201_220000_CN_377444648_220000/LConn2
  _CN_173999201_220000_CN_376502734_220000/LConn3 -- T_173999201_220000_Napoli_Levante/LConn3 -- _CN_173999201_220000_CN_377444648_220000/LConn3 -- bus132/LConn1
  _CN_173999201_220000_CN_376502734_220000/RConn1 -- T_376502734_220000_Casoria/LConn1 -- Casoria_Imi_sud_CN_377438327_220000_CN_376502734_220000/LConn1
  _CN_173999201_220000_CN_376502734_220000/RConn2 -- T_376502734_220000_Casoria/LConn2 -- Casoria_Imi_sud_CN_377438327_220000_CN_376502734_220000/LConn2
  _CN_173999201_220000_CN_376502734_220000/RConn3 -- T_376502734_220000_Casoria/LConn3 -- Casoria_Imi_sud_CN_377438327_220000_CN_376502734_220000/LConn3 -- bus133/LConn1
  _CN_173999201_220000_CN_377444648_220000/RConn1 -- T_377444648_220000_/LConn1 -- Fratta_Secondigliano_CN_377444657_220000_CN_377444648_220000/LConn1
  _CN_173999201_220000_CN_377444648_220000/RConn2 -- T_377444648_220000_/LConn2 -- Fratta_Secondigliano_CN_377444657_220000_CN_377444648_220000/LConn2
  _CN_173999201_220000_CN_377444648_220000/RConn3 -- T_377444648_220000_/LConn3 -- Fratta_Secondigliano_CN_377444657_220000_CN_377444648_220000/LConn3 -- bus134/LConn1
  Grosotto_Grosio_CN_80442466_220000_CN_165503884_220000/LConn1 -- T_80442466_220000_Grosio/LConn1 -- Grosio_Milano_Ricevitrice_Sud_CN_80442466_220000_CN163056512/LConn1 -- Grosio_Milano_Ricevitrice_Sud_CN_80442466_220000_CN_135270825_220000/RConn1
  Grosotto_Grosio_CN_80442466_220000_CN_165503884_220000/LConn2 -- T_80442466_220000_Grosio/LConn2 -- Grosio_Milano_Ricevitrice_Sud_CN_80442466_220000_CN163056512/LConn2 -- Grosio_Milano_Ricevitrice_Sud_CN_80442466_220000_CN_135270825_220000/RConn2
  Grosotto_Grosio_CN_80442466_220000_CN_165503884_220000/LConn3 -- T_80442466_220000_Grosio/LConn3 -- Grosio_Milano_Ricevitrice_Sud_CN_80442466_220000_CN163056512/LConn3 -- Grosio_Milano_Ricevitrice_Sud_CN_80442466_220000_CN_135270825_220000/RConn3 -- bus135/LConn1
  T_165503884_220000_Grosotto/LConn1 -- Grosotto_Grosio_CN_80442466_220000_CN_165503884_220000/RConn1
  T_165503884_220000_Grosotto/LConn2 -- Grosotto_Grosio_CN_80442466_220000_CN_165503884_220000/RConn2
  Grosotto_Grosio_CN_80442466_220000_CN_165503884_220000/RConn3 -- T_165503884_220000_Grosotto/LConn3 -- bus136/LConn1
  G_163056512_Centrale_idroelettrica_di_Premadio/RConn1 -- Grosio_Milano_Ricevitrice_Sud_CN_80442466_220000_CN163056512/RConn1
  G_163056512_Centrale_idroelettrica_di_Premadio/RConn2 -- Grosio_Milano_Ricevitrice_Sud_CN_80442466_220000_CN163056512/RConn2
  Grosio_Milano_Ricevitrice_Sud_CN_80442466_220000_CN163056512/RConn3 -- G_163056512_Centrale_idroelettrica_di_Premadio/RConn3 -- bus137/LConn1
  T_105757795_220000_Campochiesa/LConn1 -- Campochiesa_Camporosso_CN_105757795_220000_CN_103653567_220000/LConn1
  T_105757795_220000_Campochiesa/LConn2 -- Campochiesa_Camporosso_CN_105757795_220000_CN_103653567_220000/LConn2
  Campochiesa_Camporosso_CN_105757795_220000_CN_103653567_220000/LConn3 -- T_105757795_220000_Campochiesa/LConn3 -- bus138/LConn1
  T_103653567_220000_centrale_elettrica_di_Camporosso/LConn1 -- Campochiesa_Camporosso_CN_105757795_220000_CN_103653567_220000/RConn1
  T_103653567_220000_centrale_elettrica_di_Camporosso/LConn2 -- Campochiesa_Camporosso_CN_105757795_220000_CN_103653567_220000/RConn2
  Campochiesa_Camporosso_CN_105757795_220000_CN_103653567_220000/RConn3 -- T_103653567_220000_centrale_elettrica_di_Camporosso/LConn3 -- bus139/LConn1
  T_309371153_220000_TO_Sud/LConn1 -- _CN_309371153_220000_CN_309371152_220000/LConn1
  T_309371153_220000_TO_Sud/LConn2 -- _CN_309371153_220000_CN_309371152_220000/LConn2
  _CN_309371153_220000_CN_309371152_220000/LConn3 -- T_309371153_220000_TO_Sud/LConn3 -- bus140/LConn1
  _CN_309371153_220000_CN_309371152_220000/RConn1 -- T_309371152_220000_TO_Centro/LConn1 -- _CN_103725268_220000_CN_309371152_220000/LConn1
  _CN_309371153_220000_CN_309371152_220000/RConn2 -- T_309371152_220000_TO_Centro/LConn2 -- _CN_103725268_220000_CN_309371152_220000/LConn2
  _CN_309371153_220000_CN_309371152_220000/RConn3 -- T_309371152_220000_TO_Centro/LConn3 -- _CN_103725268_220000_CN_309371152_220000/LConn3 -- bus141/LConn1
  T_350356755_220000_Colorno/LConn1 -- Colorno_Marcaria_CN_350356755_220000_CN_163058980_220000/LConn1
  T_350356755_220000_Colorno/LConn2 -- Colorno_Marcaria_CN_350356755_220000_CN_163058980_220000/LConn2
  Colorno_Marcaria_CN_350356755_220000_CN_163058980_220000/LConn3 -- T_350356755_220000_Colorno/LConn3 -- bus142/LConn1
  Colorno_Marcaria_CN_350356755_220000_CN_163058980_220000/RConn1 -- T_163058980_220000_Marcaria/LConn1 -- Mincio_Marcaria_CN_163058980_220000_CN103562617/RConn1 -- Mincio_Marcaria_CN_163058980_220000_CN_111020792_220000/LConn1
  Colorno_Marcaria_CN_350356755_220000_CN_163058980_220000/RConn2 -- T_163058980_220000_Marcaria/LConn2 -- Mincio_Marcaria_CN_163058980_220000_CN103562617/RConn2 -- Mincio_Marcaria_CN_163058980_220000_CN_111020792_220000/LConn2
  Colorno_Marcaria_CN_350356755_220000_CN_163058980_220000/RConn3 -- T_163058980_220000_Marcaria/LConn3 -- Mincio_Marcaria_CN_163058980_220000_CN103562617/RConn3 -- Mincio_Marcaria_CN_163058980_220000_CN_111020792_220000/LConn3 -- bus143/LConn1
  Corriolo___Caracoli_Sorgente_CN_191960170_220000_CN_57736553_220000/LConn1 -- T_191960170_220000_Corriolo/LConn1 -- Corriolo_Caracoli___Sorgente_CN_191960170_220000_CN_110138220_220000/RConn1
  Corriolo___Caracoli_Sorgente_CN_191960170_220000_CN_57736553_220000/LConn2 -- T_191960170_220000_Corriolo/LConn2 -- Corriolo_Caracoli___Sorgente_CN_191960170_220000_CN_110138220_220000/RConn2
  Corriolo___Caracoli_Sorgente_CN_191960170_220000_CN_57736553_220000/LConn3 -- T_191960170_220000_Corriolo/LConn3 -- Corriolo_Caracoli___Sorgente_CN_191960170_220000_CN_110138220_220000/RConn3 -- bus144/LConn1
  Corriolo___Caracoli_Sorgente_CN_191960170_220000_CN_57736553_220000/RConn1 -- T_57736553_220000_Caracoli/LConn1 -- _CN_57736553_220000_CN_57403755_220000/LConn1 -- _CN_57736553_220000_CN53456167/LConn1 -- _CN_172705586_220000_CN_57736553_220000/LConn1
  Corriolo___Caracoli_Sorgente_CN_191960170_220000_CN_57736553_220000/RConn2 -- T_57736553_220000_Caracoli/LConn2 -- _CN_57736553_220000_CN_57403755_220000/LConn2 -- _CN_57736553_220000_CN53456167/LConn2 -- _CN_172705586_220000_CN_57736553_220000/LConn2
  Corriolo___Caracoli_Sorgente_CN_191960170_220000_CN_57736553_220000/RConn3 -- T_57736553_220000_Caracoli/LConn3 -- _CN_57736553_220000_CN_57403755_220000/LConn3 -- bus145/LConn1 -- _CN_57736553_220000_CN53456167/LConn3 -- _CN_172705586_220000_CN_57736553_220000/LConn3
  _CN_136626367_220000_CN_375892275_220000/LConn1 -- T_136626367__/LConn1 -- Samim_CN_136626367_220000_CN_375892277_220000/LConn1 -- _CN_136626367_220000_CN_375892272_220000/LConn1
  _CN_136626367_220000_CN_375892275_220000/LConn2 -- T_136626367__/LConn2 -- Samim_CN_136626367_220000_CN_375892277_220000/LConn2 -- _CN_136626367_220000_CN_375892272_220000/LConn2
  _CN_136626367_220000_CN_375892275_220000/LConn3 -- T_136626367__/LConn3 -- Samim_CN_136626367_220000_CN_375892277_220000/LConn3 -- _CN_136626367_220000_CN_375892272_220000/LConn3 -- bus146/LConn1
  T_375892275_220000_Eurallumina/LConn1 -- _CN_136626367_220000_CN_375892275_220000/RConn1
  T_375892275_220000_Eurallumina/LConn2 -- _CN_136626367_220000_CN_375892275_220000/RConn2
  _CN_136626367_220000_CN_375892275_220000/RConn3 -- T_375892275_220000_Eurallumina/LConn3 -- bus147/LConn1
  T_375892277_220000_Samim/LConn1 -- Samim_CN_136626367_220000_CN_375892277_220000/RConn1
  T_375892277_220000_Samim/LConn2 -- Samim_CN_136626367_220000_CN_375892277_220000/RConn2
  Samim_CN_136626367_220000_CN_375892277_220000/RConn3 -- T_375892277_220000_Samim/LConn3 -- bus148/LConn1
  T_375892272_220000_Samim/LConn1 -- _CN_136626367_220000_CN_375892272_220000/RConn1
  T_375892272_220000_Samim/LConn2 -- _CN_136626367_220000_CN_375892272_220000/RConn2
  _CN_136626367_220000_CN_375892272_220000/RConn3 -- T_375892272_220000_Samim/LConn3 -- bus149/LConn1
  Tavazzano_est_Cesano_Maderno_CN_107204719_220000_CN_74359510_220000/LConn1 -- T_107204719_220000_Tavazzano_Est/LConn1 -- Colà_Tavazzano_est_CN_107204719_220000_CN_156001981_220000/LConn1 -- Colà_Tavazzano_est_CN_107204719_220000_CN_116916459_220000/LConn1 -- Tavazzano_Est_Sarmato_CN_107204719_220000_CN117015784/LConn1
  Tavazzano_est_Cesano_Maderno_CN_107204719_220000_CN_74359510_220000/LConn2 -- T_107204719_220000_Tavazzano_Est/LConn2 -- Colà_Tavazzano_est_CN_107204719_220000_CN_156001981_220000/LConn2 -- Colà_Tavazzano_est_CN_107204719_220000_CN_116916459_220000/LConn2 -- Tavazzano_Est_Sarmato_CN_107204719_220000_CN117015784/LConn2
  Tavazzano_est_Cesano_Maderno_CN_107204719_220000_CN_74359510_220000/LConn3 -- T_107204719_220000_Tavazzano_Est/LConn3 -- Colà_Tavazzano_est_CN_107204719_220000_CN_156001981_220000/LConn3 -- Colà_Tavazzano_est_CN_107204719_220000_CN_116916459_220000/LConn3 -- bus150/LConn1 -- Tavazzano_Est_Sarmato_CN_107204719_220000_CN117015784/LConn3
  Tavazzano_est_Cesano_Maderno_CN_107204719_220000_CN_74359510_220000/RConn1 -- T_74359510_220000_Cesano_Maderno/LConn1 -- Cesano_Maderno_Tirano_CN_74359510_220000_CN_377832777_220000/LConn1 -- Cesano_Maderno_Tirano_CN_74359510_220000_CN_98787157_220000/LConn1
  Tavazzano_est_Cesano_Maderno_CN_107204719_220000_CN_74359510_220000/RConn2 -- T_74359510_220000_Cesano_Maderno/LConn2 -- Cesano_Maderno_Tirano_CN_74359510_220000_CN_377832777_220000/LConn2 -- Cesano_Maderno_Tirano_CN_74359510_220000_CN_98787157_220000/LConn2
  Tavazzano_est_Cesano_Maderno_CN_107204719_220000_CN_74359510_220000/RConn3 -- T_74359510_220000_Cesano_Maderno/LConn3 -- Cesano_Maderno_Tirano_CN_74359510_220000_CN_377832777_220000/LConn3 -- Cesano_Maderno_Tirano_CN_74359510_220000_CN_98787157_220000/LConn3 -- bus151/LConn1
  G_117015784_Edison/RConn1 -- Tavazzano_Est_Sarmato_CN_107204719_220000_CN117015784/RConn1
  G_117015784_Edison/RConn2 -- Tavazzano_Est_Sarmato_CN_107204719_220000_CN117015784/RConn2
  Tavazzano_Est_Sarmato_CN_107204719_220000_CN117015784/RConn3 -- G_117015784_Edison/RConn3 -- bus152/LConn1
  Colà_Tavazzano_est_CN_107204719_220000_CN_156001981_220000/RConn1 -- T_156001981_220000_Colà/LConn1 -- Sandrà_Colà_CN_156001963_220000_CN_156001981_220000/RConn1
  Colà_Tavazzano_est_CN_107204719_220000_CN_156001981_220000/RConn2 -- T_156001981_220000_Colà/LConn2 -- Sandrà_Colà_CN_156001963_220000_CN_156001981_220000/RConn2
  Colà_Tavazzano_est_CN_107204719_220000_CN_156001981_220000/RConn3 -- T_156001981_220000_Colà/LConn3 -- Sandrà_Colà_CN_156001963_220000_CN_156001981_220000/RConn3 -- bus153/LConn1
  Colà_Tavazzano_est_CN_107204719_220000_CN_116916459_220000/RConn1 -- T_116916459_220000_Tavazzano_ST/LConn1 -- Tavazzano_Ovest_Tavazzano_CN_116916459_220000_CN_107241327_220000/LConn1 -- _CN_116916459_220000_CN_162960205_220000/LConn1 -- Milano_Ricevitrice_Sud_Tavazzano_CN_116916459_220000_CN_135270825_220000/RConn1
  Colà_Tavazzano_est_CN_107204719_220000_CN_116916459_220000/RConn2 -- T_116916459_220000_Tavazzano_ST/LConn2 -- Tavazzano_Ovest_Tavazzano_CN_116916459_220000_CN_107241327_220000/LConn2 -- _CN_116916459_220000_CN_162960205_220000/LConn2 -- Milano_Ricevitrice_Sud_Tavazzano_CN_116916459_220000_CN_135270825_220000/RConn2
  Colà_Tavazzano_est_CN_107204719_220000_CN_116916459_220000/RConn3 -- T_116916459_220000_Tavazzano_ST/LConn3 -- Tavazzano_Ovest_Tavazzano_CN_116916459_220000_CN_107241327_220000/LConn3 -- bus154/LConn1 -- _CN_116916459_220000_CN_162960205_220000/LConn3 -- Milano_Ricevitrice_Sud_Tavazzano_CN_116916459_220000_CN_135270825_220000/RConn3
  Monfalcone_Rediipuglia_CN_60725872_220000_CN_41892273_220000/LConn1 -- T_60725872_380000_Monfalcone_sezione_1_220/RConn1 -- Monfalcone_Rediipuglia_CN_60725872_220000_CN_61038773_220000/LConn1
  Monfalcone_Rediipuglia_CN_60725872_220000_CN_41892273_220000/LConn2 -- T_60725872_380000_Monfalcone_sezione_1_220/RConn2 -- Monfalcone_Rediipuglia_CN_60725872_220000_CN_61038773_220000/LConn2
  Monfalcone_Rediipuglia_CN_60725872_220000_CN_41892273_220000/LConn3 -- T_60725872_380000_Monfalcone_sezione_1_220/RConn3 -- Monfalcone_Rediipuglia_CN_60725872_220000_CN_61038773_220000/LConn3 -- bus155/LConn1
  Monfalcone_Rediipuglia_CN_60725872_220000_CN_41892273_220000/RConn1 -- T_41892273_380000_Redipuglia/RConn4 -- Udine_N_E____Redipuglia_con_derivazione_Safau_CN_41892273_220000_CN_59604857_220000/LConn1
  Monfalcone_Rediipuglia_CN_60725872_220000_CN_41892273_220000/RConn2 -- T_41892273_380000_Redipuglia/RConn5 -- Udine_N_E____Redipuglia_con_derivazione_Safau_CN_41892273_220000_CN_59604857_220000/LConn2
  Monfalcone_Rediipuglia_CN_60725872_220000_CN_41892273_220000/RConn3 -- T_41892273_380000_Redipuglia/RConn6 -- Udine_N_E____Redipuglia_con_derivazione_Safau_CN_41892273_220000_CN_59604857_220000/LConn3 -- bus156/LConn1
  T_61038773_220000_Padriciano/LConn1 -- Monfalcone_Rediipuglia_CN_60725872_220000_CN_61038773_220000/RConn1
  T_61038773_220000_Padriciano/LConn2 -- Monfalcone_Rediipuglia_CN_60725872_220000_CN_61038773_220000/RConn2
  Monfalcone_Rediipuglia_CN_60725872_220000_CN_61038773_220000/RConn3 -- T_61038773_220000_Padriciano/LConn3 -- bus157/LConn1
  _CN_105141365_220000_CN_82651599_220000/LConn1 -- T_105141365_380000_Laboratori_Cesi_Chivasso/RConn4 -- _CN_105141365_220000_CN_74869121_220000/LConn1
  _CN_105141365_220000_CN_82651599_220000/LConn2 -- T_105141365_380000_Laboratori_Cesi_Chivasso/RConn5 -- _CN_105141365_220000_CN_74869121_220000/LConn2
  _CN_105141365_220000_CN_82651599_220000/LConn3 -- T_105141365_380000_Laboratori_Cesi_Chivasso/RConn6 -- _CN_105141365_220000_CN_74869121_220000/LConn3 -- bus158/LConn1
  _CN_105141365_220000_CN_82651599_220000/RConn1 -- T_82651599_220000_Biella_Est/LConn1 -- Biella_Est___Turbigo_CN_162828577_220000_CN_82651599_220000/LConn1
  _CN_105141365_220000_CN_82651599_220000/RConn2 -- T_82651599_220000_Biella_Est/LConn2 -- Biella_Est___Turbigo_CN_162828577_220000_CN_82651599_220000/LConn2
  _CN_105141365_220000_CN_82651599_220000/RConn3 -- T_82651599_220000_Biella_Est/LConn3 -- Biella_Est___Turbigo_CN_162828577_220000_CN_82651599_220000/LConn3 -- bus159/LConn1
  _CN_105141365_220000_CN_74869121_220000/RConn1 -- T_74869121_380000_Rondissone/RConn4 -- _CN_74869121_220000_CN_105153431_220000/LConn1 -- Chivasso_Termica___Rondissone_CN_102287716_220000_CN_74869121_220000/LConn1
  _CN_105141365_220000_CN_74869121_220000/RConn2 -- T_74869121_380000_Rondissone/RConn5 -- _CN_74869121_220000_CN_105153431_220000/LConn2 -- Chivasso_Termica___Rondissone_CN_102287716_220000_CN_74869121_220000/LConn2
  _CN_105141365_220000_CN_74869121_220000/RConn3 -- T_74869121_380000_Rondissone/RConn6 -- _CN_74869121_220000_CN_105153431_220000/LConn3 -- bus160/LConn1 -- Chivasso_Termica___Rondissone_CN_102287716_220000_CN_74869121_220000/LConn3
  _CN_99826025_220000_CN_103725268_220000/RConn1 -- T_103725268_220000_Stura/LConn1 -- _CN_103725268_220000_CN_309371152_220000/RConn1 -- Stura_Sondel_CN_103725268_220000_CN_103725446_220000/LConn1
  _CN_99826025_220000_CN_103725268_220000/RConn2 -- T_103725268_220000_Stura/LConn2 -- _CN_103725268_220000_CN_309371152_220000/RConn2 -- Stura_Sondel_CN_103725268_220000_CN_103725446_220000/LConn2
  _CN_99826025_220000_CN_103725268_220000/RConn3 -- T_103725268_220000_Stura/LConn3 -- _CN_103725268_220000_CN_309371152_220000/RConn3 -- bus161/LConn1 -- Stura_Sondel_CN_103725268_220000_CN_103725446_220000/LConn3
  Vignole_Borbera___Casanova_CN_99826025_220000_CN_100952845_220000/RConn1 -- T_100952845_380000_Vignole/RConn4 -- Vignole_Ilva_CN_101346508_220000_CN_100952845_220000/LConn1 -- Vignole___San_Colombano_CN_103653565_220000_CN_100952845_220000/LConn1 -- Morigallo_Vignole_CN_61484190_220000_CN_100952845_220000/RConn1
  Vignole_Borbera___Casanova_CN_99826025_220000_CN_100952845_220000/RConn2 -- T_100952845_380000_Vignole/RConn5 -- Vignole_Ilva_CN_101346508_220000_CN_100952845_220000/LConn2 -- Vignole___San_Colombano_CN_103653565_220000_CN_100952845_220000/LConn2 -- Morigallo_Vignole_CN_61484190_220000_CN_100952845_220000/RConn2
  Vignole_Borbera___Casanova_CN_99826025_220000_CN_100952845_220000/RConn3 -- T_100952845_380000_Vignole/RConn6 -- Vignole_Ilva_CN_101346508_220000_CN_100952845_220000/LConn3 -- bus162/LConn1 -- Vignole___San_Colombano_CN_103653565_220000_CN_100952845_220000/LConn3 -- Morigallo_Vignole_CN_61484190_220000_CN_100952845_220000/RConn3
  _CN_79879290_220000_CN_68299044_220000/RConn1 -- T_79879290_220000_Ricevitrice_Nord_Milano/LConn1 -- _CN_79879290_220000_CN_79879307_220000/RConn1 -- _CN_79879290_220000_CN67400512/RConn1
  _CN_79879290_220000_CN_68299044_220000/RConn2 -- T_79879290_220000_Ricevitrice_Nord_Milano/LConn2 -- _CN_79879290_220000_CN_79879307_220000/RConn2 -- _CN_79879290_220000_CN67400512/RConn2
  _CN_79879290_220000_CN_68299044_220000/RConn3 -- T_79879290_220000_Ricevitrice_Nord_Milano/LConn3 -- _CN_79879290_220000_CN_79879307_220000/RConn3 -- _CN_79879290_220000_CN67400512/RConn3 -- bus163/LConn1
  T_146652798_220000_Centro_Energia_Teverola/LConn1 -- Aversa_Centro_Energia_Teverola_CN_146652798_220000_CN_132701980_220000/LConn1
  T_146652798_220000_Centro_Energia_Teverola/LConn2 -- Aversa_Centro_Energia_Teverola_CN_146652798_220000_CN_132701980_220000/LConn2
  Aversa_Centro_Energia_Teverola_CN_146652798_220000_CN_132701980_220000/LConn3 -- T_146652798_220000_Centro_Energia_Teverola/LConn3 -- bus164/LConn1
  Aversa_Centro_Energia_Teverola_CN_146652798_220000_CN_132701980_220000/RConn1 -- T_132701980_220000_Aversa/LConn1 -- Aversa_Fratta_CN_132701980_220000_CN_132702940_220000/RConn1 -- Aversa_Santa_Maria_Capua_Vetere_CN_132701980_220000_CN_93860115_220000/LConn1
  Aversa_Centro_Energia_Teverola_CN_146652798_220000_CN_132701980_220000/RConn2 -- T_132701980_220000_Aversa/LConn2 -- Aversa_Fratta_CN_132701980_220000_CN_132702940_220000/RConn2 -- Aversa_Santa_Maria_Capua_Vetere_CN_132701980_220000_CN_93860115_220000/LConn2
  Aversa_Centro_Energia_Teverola_CN_146652798_220000_CN_132701980_220000/RConn3 -- T_132701980_220000_Aversa/LConn3 -- Aversa_Fratta_CN_132701980_220000_CN_132702940_220000/RConn3 -- Aversa_Santa_Maria_Capua_Vetere_CN_132701980_220000_CN_93860115_220000/LConn3 -- bus165/LConn1
  Borgo_Valsugana_Lavis_CN_96658563_220000_CN_103549584_220000/LConn1 -- T_96658563_220000_Lavis/LConn1 -- Lavis_Trento_sud_CN_96658563_220000_CN_147466201_220000/RConn1 -- Lavis_San_Floriano_CN_96658563_220000_CN_151070909_220000/LConn1
  Borgo_Valsugana_Lavis_CN_96658563_220000_CN_103549584_220000/LConn2 -- T_96658563_220000_Lavis/LConn2 -- Lavis_Trento_sud_CN_96658563_220000_CN_147466201_220000/RConn2 -- Lavis_San_Floriano_CN_96658563_220000_CN_151070909_220000/LConn2
  Borgo_Valsugana_Lavis_CN_96658563_220000_CN_103549584_220000/LConn3 -- T_96658563_220000_Lavis/LConn3 -- Lavis_Trento_sud_CN_96658563_220000_CN_147466201_220000/RConn3 -- bus166/LConn1 -- Lavis_San_Floriano_CN_96658563_220000_CN_151070909_220000/LConn3
  Borgo_Valsugana_Lavis_CN_96658563_220000_CN_103549584_220000/RConn1 -- T_103549584_220000_Borgo_Valsugana/LConn1 -- _CN_214294769_220000_CN_103549584_220000/LConn1 -- Borgo_Valsugana_Acciaieria_CN_103549584_220000_CN_149071351_220000/LConn1
  Borgo_Valsugana_Lavis_CN_96658563_220000_CN_103549584_220000/RConn2 -- T_103549584_220000_Borgo_Valsugana/LConn2 -- _CN_214294769_220000_CN_103549584_220000/LConn2 -- Borgo_Valsugana_Acciaieria_CN_103549584_220000_CN_149071351_220000/LConn2
  Borgo_Valsugana_Lavis_CN_96658563_220000_CN_103549584_220000/RConn3 -- T_103549584_220000_Borgo_Valsugana/LConn3 -- _CN_214294769_220000_CN_103549584_220000/LConn3 -- Borgo_Valsugana_Acciaieria_CN_103549584_220000_CN_149071351_220000/LConn3 -- bus167/LConn1
  Lavis_San_Floriano_CN_96658563_220000_CN_151070909_220000/RConn1 -- T_151070909_220000_San_Floriano_d'Egna/LConn1 -- _CN_35680992_220000_CN_151070909_220000/LConn1
  Lavis_San_Floriano_CN_96658563_220000_CN_151070909_220000/RConn2 -- T_151070909_220000_San_Floriano_d'Egna/LConn2 -- _CN_35680992_220000_CN_151070909_220000/LConn2
  Lavis_San_Floriano_CN_96658563_220000_CN_151070909_220000/RConn3 -- T_151070909_220000_San_Floriano_d'Egna/LConn3 -- _CN_35680992_220000_CN_151070909_220000/LConn3 -- bus168/LConn1
  Presenzano_Santa_Maria_Capua_Vetere_CN_419423704_220000_CN83246343/LConn1 -- T_419423704_220000_Presenzano_TR/LConn1 -- Presenzano_Santa_Maria_Capua_Vetere_CN_419423704_220000_CN_93860115_220000/LConn1
  Presenzano_Santa_Maria_Capua_Vetere_CN_419423704_220000_CN83246343/LConn2 -- T_419423704_220000_Presenzano_TR/LConn2 -- Presenzano_Santa_Maria_Capua_Vetere_CN_419423704_220000_CN_93860115_220000/LConn2
  Presenzano_Santa_Maria_Capua_Vetere_CN_419423704_220000_CN83246343/LConn3 -- T_419423704_220000_Presenzano_TR/LConn3 -- Presenzano_Santa_Maria_Capua_Vetere_CN_419423704_220000_CN_93860115_220000/LConn3 -- bus169/LConn1
  Presenzano_Santa_Maria_Capua_Vetere_CN_419423704_220000_CN83246343/RConn1 -- G_83246343_Centrale_di_Capriati_al_Volturno/RConn1 -- Popoli_Capriati_CN_84277460_220000_CN83246343/LConn1
  Presenzano_Santa_Maria_Capua_Vetere_CN_419423704_220000_CN83246343/RConn2 -- G_83246343_Centrale_di_Capriati_al_Volturno/RConn2 -- Popoli_Capriati_CN_84277460_220000_CN83246343/LConn2
  Presenzano_Santa_Maria_Capua_Vetere_CN_419423704_220000_CN83246343/RConn3 -- G_83246343_Centrale_di_Capriati_al_Volturno/RConn3 -- Popoli_Capriati_CN_84277460_220000_CN83246343/LConn3 -- bus170/LConn1
  Presenzano_Santa_Maria_Capua_Vetere_CN_419423704_220000_CN_93860115_220000/RConn1 -- T_93860115_380000_Santa_Maria_Capua_Vetere/RConn4 -- Aversa_Santa_Maria_Capua_Vetere_CN_132701980_220000_CN_93860115_220000/RConn1
  Presenzano_Santa_Maria_Capua_Vetere_CN_419423704_220000_CN_93860115_220000/RConn2 -- T_93860115_380000_Santa_Maria_Capua_Vetere/RConn5 -- Aversa_Santa_Maria_Capua_Vetere_CN_132701980_220000_CN_93860115_220000/RConn2
  Presenzano_Santa_Maria_Capua_Vetere_CN_419423704_220000_CN_93860115_220000/RConn3 -- T_93860115_380000_Santa_Maria_Capua_Vetere/RConn6 -- Aversa_Santa_Maria_Capua_Vetere_CN_132701980_220000_CN_93860115_220000/RConn3 -- bus171/LConn1
  T_202772821_220000_Ganda/LConn1 -- Belviso_Ganda_CN_202772821_220000_CN163056519/RConn1
  T_202772821_220000_Ganda/LConn2 -- Belviso_Ganda_CN_202772821_220000_CN163056519/RConn2
  Belviso_Ganda_CN_202772821_220000_CN163056519/RConn3 -- T_202772821_220000_Ganda/LConn3 -- bus172/LConn1
  T_61375111_380000_Villanova/RConn4 -- Montorio_Villanova_CN_61375111_220000_CN_158652469_220000/RConn1
  T_61375111_380000_Villanova/RConn5 -- Montorio_Villanova_CN_61375111_220000_CN_158652469_220000/RConn2
  Montorio_Villanova_CN_61375111_220000_CN_158652469_220000/RConn3 -- T_61375111_380000_Villanova/RConn6 -- bus173/LConn1
  _CN_139758444_220000_CN_139442467_220000/LConn1 -- T_139758444_220000_Querceto/LConn1 -- _CN_139758444_220000_CN_40634284_220000/LConn1
  _CN_139758444_220000_CN_139442467_220000/LConn2 -- T_139758444_220000_Querceto/LConn2 -- _CN_139758444_220000_CN_40634284_220000/LConn2
  _CN_139758444_220000_CN_139442467_220000/LConn3 -- T_139758444_220000_Querceto/LConn3 -- _CN_139758444_220000_CN_40634284_220000/LConn3 -- bus174/LConn1
  T_139442467_380000_Colunga/RConn4 -- _CN_139758444_220000_CN_139442467_220000/RConn1
  T_139442467_380000_Colunga/RConn5 -- _CN_139758444_220000_CN_139442467_220000/RConn2
  _CN_139758444_220000_CN_139442467_220000/RConn3 -- T_139442467_380000_Colunga/RConn6 -- bus175/LConn1
  T_40634284_380000_Calenzano/RConn4 -- _CN_139758444_220000_CN_40634284_220000/RConn1
  T_40634284_380000_Calenzano/RConn5 -- _CN_139758444_220000_CN_40634284_220000/RConn2
  _CN_139758444_220000_CN_40634284_220000/RConn3 -- T_40634284_380000_Calenzano/RConn6 -- bus176/LConn1
  Cassano_Tavazzano_Ovest_CN_75947658_220000_CN_107241327_220000/RConn1 -- T_107241327_220000_Tavazzano_Ovest/LConn1 -- Tavazzano_Ovest_Tavazzano_CN_116916459_220000_CN_107241327_220000/RConn1
  Cassano_Tavazzano_Ovest_CN_75947658_220000_CN_107241327_220000/RConn2 -- T_107241327_220000_Tavazzano_Ovest/LConn2 -- Tavazzano_Ovest_Tavazzano_CN_116916459_220000_CN_107241327_220000/RConn2
  Cassano_Tavazzano_Ovest_CN_75947658_220000_CN_107241327_220000/RConn3 -- T_107241327_220000_Tavazzano_Ovest/LConn3 -- Tavazzano_Ovest_Tavazzano_CN_116916459_220000_CN_107241327_220000/RConn3 -- bus177/LConn1
  T_203468251_220000;132000_RISE_Sesto/LConn1 -- _CN_75947658_220000_CN_203468251_220000/RConn1
  T_203468251_220000;132000_RISE_Sesto/LConn2 -- _CN_75947658_220000_CN_203468251_220000/RConn2
  _CN_75947658_220000_CN_203468251_220000/RConn3 -- T_203468251_220000;132000_RISE_Sesto/LConn3 -- bus178/LConn1
  Fratta_Poggioreale_CN_93850768_220000_CN_132702940_220000/RConn1 -- T_93850768_220000_Castelluccia/LConn1 -- San_Sebastiano_Castelluccia_CN_93850768_220000_CN_202179289_220000/LConn1 -- Castelluccia_Casalnuovo_CN_93850768_220000_CN_370679021_220000/RConn1
  Fratta_Poggioreale_CN_93850768_220000_CN_132702940_220000/RConn2 -- T_93850768_220000_Castelluccia/LConn2 -- San_Sebastiano_Castelluccia_CN_93850768_220000_CN_202179289_220000/LConn2 -- Castelluccia_Casalnuovo_CN_93850768_220000_CN_370679021_220000/RConn2
  Fratta_Poggioreale_CN_93850768_220000_CN_132702940_220000/RConn3 -- T_93850768_220000_Castelluccia/LConn3 -- San_Sebastiano_Castelluccia_CN_93850768_220000_CN_202179289_220000/LConn3 -- Castelluccia_Casalnuovo_CN_93850768_220000_CN_370679021_220000/RConn3 -- bus179/LConn1
  San_Sebastiano_Castelluccia_CN_93850768_220000_CN_202179289_220000/RConn1 -- T_202179289_220000_/LConn1 -- San_Sebastiano_Castelluccia_CN_202179289_220000_CN_202179060_220000/RConn1
  San_Sebastiano_Castelluccia_CN_93850768_220000_CN_202179289_220000/RConn2 -- T_202179289_220000_/LConn2 -- San_Sebastiano_Castelluccia_CN_202179289_220000_CN_202179060_220000/RConn2
  San_Sebastiano_Castelluccia_CN_93850768_220000_CN_202179289_220000/RConn3 -- T_202179289_220000_/LConn3 -- San_Sebastiano_Castelluccia_CN_202179289_220000_CN_202179060_220000/RConn3 -- bus180/LConn1
  T_59604857_220000_Acciaieria_Bertoli/LConn1 -- Udine_N_E____Redipuglia_con_derivazione_Safau_CN_41892273_220000_CN_59604857_220000/RConn1
  T_59604857_220000_Acciaieria_Bertoli/LConn2 -- Udine_N_E____Redipuglia_con_derivazione_Safau_CN_41892273_220000_CN_59604857_220000/RConn2
  Udine_N_E____Redipuglia_con_derivazione_Safau_CN_41892273_220000_CN_59604857_220000/RConn3 -- T_59604857_220000_Acciaieria_Bertoli/LConn3 -- bus181/LConn1
  _CN_165371026_220000_CN_165371027_220000/RConn1 -- T_165371027__/LConn1 -- SantaLucia_Roma_Nord_2_CN_165371027_220000_CN_82762493_220000/LConn1
  _CN_165371026_220000_CN_165371027_220000/RConn2 -- T_165371027__/LConn2 -- SantaLucia_Roma_Nord_2_CN_165371027_220000_CN_82762493_220000/LConn2
  _CN_165371026_220000_CN_165371027_220000/RConn3 -- T_165371027__/LConn3 -- SantaLucia_Roma_Nord_2_CN_165371027_220000_CN_82762493_220000/LConn3 -- bus182/LConn1
  SantaLucia_Roma_Nord_2_CN_165371027_220000_CN_82762493_220000/RConn1 -- T_82762493_380000_Santa_Lucia/RConn4 -- Torrevaldaliga_Sud_Santa_Lucia_CN_82762493_220000_CN_82767145_220000/LConn1
  SantaLucia_Roma_Nord_2_CN_165371027_220000_CN_82762493_220000/RConn2 -- T_82762493_380000_Santa_Lucia/RConn5 -- Torrevaldaliga_Sud_Santa_Lucia_CN_82762493_220000_CN_82767145_220000/LConn2
  SantaLucia_Roma_Nord_2_CN_165371027_220000_CN_82762493_220000/RConn3 -- T_82762493_380000_Santa_Lucia/RConn6 -- Torrevaldaliga_Sud_Santa_Lucia_CN_82762493_220000_CN_82767145_220000/LConn3 -- bus183/LConn1
  T_151205012_220000_Boazzo/LConn1 -- Cimego_TR_Boazzo_CN_151205012_220000_CN_151199514_220000/LConn1
  T_151205012_220000_Boazzo/LConn2 -- Cimego_TR_Boazzo_CN_151205012_220000_CN_151199514_220000/LConn2
  Cimego_TR_Boazzo_CN_151205012_220000_CN_151199514_220000/LConn3 -- T_151205012_220000_Boazzo/LConn3 -- bus184/LConn1
  T_151199514_220000_Cimego_TR/LConn1 -- Cimego_TR_Boazzo_CN_151205012_220000_CN_151199514_220000/RConn1
  T_151199514_220000_Cimego_TR/LConn2 -- Cimego_TR_Boazzo_CN_151205012_220000_CN_151199514_220000/RConn2
  Cimego_TR_Boazzo_CN_151205012_220000_CN_151199514_220000/RConn3 -- T_151199514_220000_Cimego_TR/LConn3 -- bus185/LConn1
  Morigallo_San_Colombano_Certenoli_CN_61484190_220000_CN_103653565_220000/RConn1 -- T_103653565_220000_San_Colombano/LConn1 -- Vignole___San_Colombano_CN_103653565_220000_CN_100952845_220000/RConn1
  Morigallo_San_Colombano_Certenoli_CN_61484190_220000_CN_103653565_220000/RConn2 -- T_103653565_220000_San_Colombano/LConn2 -- Vignole___San_Colombano_CN_103653565_220000_CN_100952845_220000/RConn2
  Morigallo_San_Colombano_Certenoli_CN_61484190_220000_CN_103653565_220000/RConn3 -- T_103653565_220000_San_Colombano/LConn3 -- Vignole___San_Colombano_CN_103653565_220000_CN_100952845_220000/RConn3 -- bus186/LConn1
  T_158599954_220000_Stazione_elettrica_di_Avenza/LConn1 -- Morigallo_San_Colombano_Certenoli_CN_61484190_220000_CN_158599954_220000/RConn1
  T_158599954_220000_Stazione_elettrica_di_Avenza/LConn2 -- Morigallo_San_Colombano_Certenoli_CN_61484190_220000_CN_158599954_220000/RConn2
  Morigallo_San_Colombano_Certenoli_CN_61484190_220000_CN_158599954_220000/RConn3 -- T_158599954_220000_Stazione_elettrica_di_Avenza/LConn3 -- bus187/LConn1
  Morigallo_Savona_CN_61484190_220000_CN_296141722_220000/RConn1 -- T_296141722_220000_Savona_T5/LConn1 -- Savona_Vado_Ligure_CN_103653591_220000_CN_296141722_220000/LConn1
  Morigallo_Savona_CN_61484190_220000_CN_296141722_220000/RConn2 -- T_296141722_220000_Savona_T5/LConn2 -- Savona_Vado_Ligure_CN_103653591_220000_CN_296141722_220000/LConn2
  Morigallo_Savona_CN_61484190_220000_CN_296141722_220000/RConn3 -- T_296141722_220000_Savona_T5/LConn3 -- Savona_Vado_Ligure_CN_103653591_220000_CN_296141722_220000/LConn3 -- bus188/LConn1
  T_375908008_220000_Fulgatore/LConn1 -- Fulgatore_Partanna_CN_375908008_220000_CN_53635045_220000/LConn1
  T_375908008_220000_Fulgatore/LConn2 -- Fulgatore_Partanna_CN_375908008_220000_CN_53635045_220000/LConn2
  Fulgatore_Partanna_CN_375908008_220000_CN_53635045_220000/LConn3 -- T_375908008_220000_Fulgatore/LConn3 -- bus189/LConn1
  Fulgatore_Partanna_CN_375908008_220000_CN_53635045_220000/RConn1 -- T_53635045__Partanna/LConn1 -- _CN_375916035_220000_CN_53635045_220000/LConn1 -- _CN_57736541_220000_CN_53635045_220000/LConn1
  Fulgatore_Partanna_CN_375908008_220000_CN_53635045_220000/RConn2 -- T_53635045__Partanna/LConn2 -- _CN_375916035_220000_CN_53635045_220000/LConn2 -- _CN_57736541_220000_CN_53635045_220000/LConn2
  Fulgatore_Partanna_CN_375908008_220000_CN_53635045_220000/RConn3 -- T_53635045__Partanna/LConn3 -- _CN_375916035_220000_CN_53635045_220000/LConn3 -- _CN_57736541_220000_CN_53635045_220000/LConn3 -- bus190/LConn1
  T_110140586_220000_San_Filippo_del_Mela_gruppi_5_e_6/LConn1 -- _CN_110140586_220000_CN139107362/RConn1
  T_110140586_220000_San_Filippo_del_Mela_gruppi_5_e_6/LConn2 -- _CN_110140586_220000_CN139107362/RConn2
  _CN_110140586_220000_CN139107362/RConn3 -- T_110140586_220000_San_Filippo_del_Mela_gruppi_5_e_6/LConn3 -- bus191/LConn1
  Sandrà_Bussolengo_CN_156001963_220000_CN_111020792_220000/RConn1 -- T_111020792_220000_Stazione_elettrica_di_Bussolengo/LConn1 -- _CN_111020792_220000_CN_162066058_220000/LConn1 -- _CN_111020792_220000_CN_59556712_220000/LConn1 -- _CN_111020792_220000_CN_289178949_220000/LConn1 -- Mincio_Marcaria_CN_163058980_220000_CN_111020792_220000/RConn1 -- Bussolengo_Ferrara_CN_111020792_220000_CN_181125039_220000/LConn1 -- Santa_Massenza_Bussolengo_CN_111020792_220000_CN_147466201_220000/RConn1 -- Mincio_Colunga_CN_111020792_220000_CN_82078641_220000/LConn1
  Sandrà_Bussolengo_CN_156001963_220000_CN_111020792_220000/RConn2 -- T_111020792_220000_Stazione_elettrica_di_Bussolengo/LConn2 -- _CN_111020792_220000_CN_162066058_220000/LConn2 -- _CN_111020792_220000_CN_59556712_220000/LConn2 -- _CN_111020792_220000_CN_289178949_220000/LConn2 -- Mincio_Marcaria_CN_163058980_220000_CN_111020792_220000/RConn2 -- Bussolengo_Ferrara_CN_111020792_220000_CN_181125039_220000/LConn2 -- Santa_Massenza_Bussolengo_CN_111020792_220000_CN_147466201_220000/RConn2 -- Mincio_Colunga_CN_111020792_220000_CN_82078641_220000/LConn2
  Sandrà_Bussolengo_CN_156001963_220000_CN_111020792_220000/RConn3 -- T_111020792_220000_Stazione_elettrica_di_Bussolengo/LConn3 -- _CN_111020792_220000_CN_162066058_220000/LConn3 -- _CN_111020792_220000_CN_59556712_220000/LConn3 -- _CN_111020792_220000_CN_289178949_220000/LConn3 -- bus192/LConn1 -- Mincio_Marcaria_CN_163058980_220000_CN_111020792_220000/RConn3 -- Bussolengo_Ferrara_CN_111020792_220000_CN_181125039_220000/LConn3 -- Santa_Massenza_Bussolengo_CN_111020792_220000_CN_147466201_220000/RConn3 -- Mincio_Colunga_CN_111020792_220000_CN_82078641_220000/LConn3
  Sandrà_Dugale_CN_156001963_220000_CN_59556712_220000/RConn1 -- T_59556712_380000_Dugale/RConn4 -- _CN_111020792_220000_CN_59556712_220000/RConn1
  Sandrà_Dugale_CN_156001963_220000_CN_59556712_220000/RConn2 -- T_59556712_380000_Dugale/RConn5 -- _CN_111020792_220000_CN_59556712_220000/RConn2
  Sandrà_Dugale_CN_156001963_220000_CN_59556712_220000/RConn3 -- T_59556712_380000_Dugale/RConn6 -- _CN_111020792_220000_CN_59556712_220000/RConn3 -- bus193/LConn1
  T_412909650_220000_Mantova_220/LConn1 -- Sandrà_Mantova_CN_156001963_220000_CN_412909650_220000/RConn1
  T_412909650_220000_Mantova_220/LConn2 -- Sandrà_Mantova_CN_156001963_220000_CN_412909650_220000/RConn2
  Sandrà_Mantova_CN_156001963_220000_CN_412909650_220000/RConn3 -- T_412909650_220000_Mantova_220/LConn3 -- bus194/LConn1
  _CN_155976563_220000_CN_155976582_220000/RConn1 -- T_155976563_220000_Conegliano/LConn1 -- _CN_155976563_220000_CN_59026315_220000/RConn1
  _CN_155976563_220000_CN_155976582_220000/RConn2 -- T_155976563_220000_Conegliano/LConn2 -- _CN_155976563_220000_CN_59026315_220000/RConn2
  _CN_155976563_220000_CN_155976582_220000/RConn3 -- T_155976563_220000_Conegliano/LConn3 -- _CN_155976563_220000_CN_59026315_220000/RConn3 -- bus195/LConn1
  Popoli_San_Giacomo_220_CN_96188601_220000_CN_84277460_220000/LConn1 -- T_96188601_220000_San_Giacomo_220/LConn1 -- _CN_96188601_220000_CN_96190189_220000/LConn1
  Popoli_San_Giacomo_220_CN_96188601_220000_CN_84277460_220000/LConn2 -- T_96188601_220000_San_Giacomo_220/LConn2 -- _CN_96188601_220000_CN_96190189_220000/LConn2
  Popoli_San_Giacomo_220_CN_96188601_220000_CN_84277460_220000/LConn3 -- T_96188601_220000_San_Giacomo_220/LConn3 -- _CN_96188601_220000_CN_96190189_220000/LConn3 -- bus196/LConn1
  Popoli_San_Giacomo_220_CN_96188601_220000_CN_84277460_220000/RConn1 -- T_84277460_220000_Popoli/LConn1 -- Popoli_Capriati_CN_84277460_220000_CN83246343/RConn1
  Popoli_San_Giacomo_220_CN_96188601_220000_CN_84277460_220000/RConn2 -- T_84277460_220000_Popoli/LConn2 -- Popoli_Capriati_CN_84277460_220000_CN83246343/RConn2
  Popoli_San_Giacomo_220_CN_96188601_220000_CN_84277460_220000/RConn3 -- T_84277460_220000_Popoli/LConn3 -- Popoli_Capriati_CN_84277460_220000_CN83246343/RConn3 -- bus197/LConn1
  T_96190189_380000_San_Giacomo_380/RConn4 -- _CN_96188601_220000_CN_96190189_220000/RConn1
  T_96190189_380000_San_Giacomo_380/RConn5 -- _CN_96188601_220000_CN_96190189_220000/RConn2
  _CN_96188601_220000_CN_96190189_220000/RConn3 -- T_96190189_380000_San_Giacomo_380/RConn6 -- bus198/LConn1
  T_108020416_380000_Laino/RConn4 -- Laino_Rotonda_CN_108020416_220000_CN_108020695_220000/RConn1
  T_108020416_380000_Laino/RConn5 -- Laino_Rotonda_CN_108020416_220000_CN_108020695_220000/RConn2
  Laino_Rotonda_CN_108020416_220000_CN_108020695_220000/RConn3 -- T_108020416_380000_Laino/RConn6 -- bus199/LConn1
  _CN_144378054_220000_CN_120916823_220000/LConn1 -- T_144378054_220000_Arezzo_C/LConn1 -- _CN_144378054_220000_CN113684324/LConn1
  _CN_144378054_220000_CN_120916823_220000/LConn2 -- T_144378054_220000_Arezzo_C/LConn2 -- _CN_144378054_220000_CN113684324/LConn2
  _CN_144378054_220000_CN_120916823_220000/LConn3 -- T_144378054_220000_Arezzo_C/LConn3 -- _CN_144378054_220000_CN113684324/LConn3 -- bus200/LConn1
  T_120916823_220000_Pietrafitta_220/LConn1 -- _CN_144378054_220000_CN_120916823_220000/RConn1
  T_120916823_220000_Pietrafitta_220/LConn2 -- _CN_144378054_220000_CN_120916823_220000/RConn2
  _CN_144378054_220000_CN_120916823_220000/RConn3 -- T_120916823_220000_Pietrafitta_220/LConn3 -- bus201/LConn1
  "G_113684324_Centrale_termoelettrica_\"Santa_Barbara\""/RConn1 -- _CN_144378054_220000_CN113684324/RConn1
  "G_113684324_Centrale_termoelettrica_\"Santa_Barbara\""/RConn2 -- _CN_144378054_220000_CN113684324/RConn2
  _CN_144378054_220000_CN113684324/RConn3 -- "G_113684324_Centrale_termoelettrica_\"Santa_Barbara\""/RConn3 -- bus202/LConn1
  T_59620552_220000_Naturno/LConn1 -- _CN_59620552_220000_CN_35680992_220000/LConn1
  T_59620552_220000_Naturno/LConn2 -- _CN_59620552_220000_CN_35680992_220000/LConn2
  _CN_59620552_220000_CN_35680992_220000/LConn3 -- T_59620552_220000_Naturno/LConn3 -- bus203/LConn1
  _CN_59620552_220000_CN_35680992_220000/RConn1 -- T_35680992_220000_Ponte_Resia/LConn1 -- _CN_35680992_220000_CN_151070909_220000/RConn1
  _CN_59620552_220000_CN_35680992_220000/RConn2 -- T_35680992_220000_Ponte_Resia/LConn2 -- _CN_35680992_220000_CN_151070909_220000/RConn2
  _CN_59620552_220000_CN_35680992_220000/RConn3 -- T_35680992_220000_Ponte_Resia/LConn3 -- _CN_35680992_220000_CN_151070909_220000/RConn3 -- bus204/LConn1
  T_101346507_220000_Novi_Ligure/LConn1 -- _CN_101346507_220000_CN_101346508_220000/LConn1
  T_101346507_220000_Novi_Ligure/LConn2 -- _CN_101346507_220000_CN_101346508_220000/LConn2
  _CN_101346507_220000_CN_101346508_220000/LConn3 -- T_101346507_220000_Novi_Ligure/LConn3 -- bus205/LConn1
